simulink library "MCHP_Blockset"  (R2014b)
settings: Solver=ode45  SolverMode=SingleTasking  StartTime=0.0  StopTime=10.0  RelTol=1e-3
InitFcn:
  | disp('MCHP_Blockset_Library_InitFunction');
undefined symbols (not defined in the file): A0, A2, AD0, AVdd, B1, B5, B9, C10, C2, CMP2A, CMP3A, CMP4A, EXTREF1, EXTREF2, gcbh, MaxPer, MCHP_ACC_SAMx_Callback, MCHP_ADC_Callback, MCHP_ADC_HighSpeed_SAR_Callback, MCHP_ADC_HighSpeed_SAR_dsPIC_Callback, MCHP_ADC_SAME5x_Callback, MCHP_AFEC_SAM7x_Callback, MCHP_BUS_I2C_MASTER_callback, MCHP_BUS_SPI_callback, MCHP_C_function_Call_callback, MCHP_CN_Callback, MCHP_COMPARATOR1_callback, MCHP_CompilerOptimisation_Callback, MCHP_DACC_SAMx_Callback, MCHP_Digital_Input_Callback, MCHP_Digital_Output_Read_Callback, MCHP_Digital_Output_Write_Callback, MCHP_Fun, MCHP_HighSpeed_AnalogComparator_Callback, MCHP_IC_Callback, MCHP_IdleTask_Callback, MCHP_Interrupt_Callback, MCHP_Master_Callback, MCHP_MCPWM_Callback, MCHP_MCU_LOAD_Callback, MCHP_MCU_OVERLOAD_Callback, MCHP_MSI_Callback, MCHP_OC_HW_Callback, MCHP_OC_SW_Callback, MCHP_OP_AMP_Callback, MCHP_OrderInOut, MCHP_PDEC_Callback, MCHP_PGA_Callback, MCHP_PWM_Callback, MCHP_PWM_HighSpeed_Override_Callback, MCHP_PWM_HS_FEP_Callback, MCHP_PWM_SAM7x_Callback, MCHP_PWM_SAM7x_Override_Callback, MCHP_QDEC_SAMx_Callback, MCHP_QEI_Callback, MCHP_Scheduler_Options_Callback, MCHP_SECONDARY_CORE_Callback, MCHP_Tasks_State_Callback, MCHP_TCC_PWM_Callback, MCHP_TIMER_Config_Callback ... (+18)
libraries: MCHP_Blockset x2
(part 8 of 9)

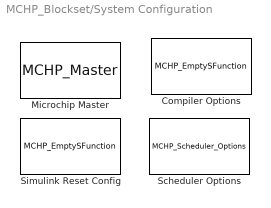
== system MCHP_Blockset/System Configuration ==
  Compiler Options : S-Function  Priority=1  InitFcn=MCHP_CompilerOptimisation_Callback(gcbh, 'InitFcn');  FunctionName=MCHP_EmptySFunction  EnableBusSupport=off  mask{LATEST_CMPLR=on, COMP_LIST=Dynamic Options, COMP_LIST_TXT=Dynamic Options, DFP_LIST=Dynamic Options, DFP_LIST_TXT=Dynamic Options, CMSIS_DSP=Dynamic Options, CMSIS_DSP_TXT=Dynamic Options, USE_64BIT_DOUBLE=off, MCHP_MULTITHREAD_COMPILATION=on, UseCustom_LinkerScript=off, LinkerScript=, MCHP_MASTERLINK=CVLK_SAME70_Modified_CompilerBlock_R2014b/Microchip Master, OPTIMIZATION_LEVEL=2, MPLAB_LINKLIB=default, MPLAB_LINKLIB1=fast floating-point math, CodeReplacement=Dynamic Options, CodeReplacement_TXT=None, OPTIMIZATION_FLTO=off, OPTIMIZATION_REORDER=off, UNROLL_LOOPS=off, PROCEDURAL_ABSTRACTION=off, CUSTOM_OPTIM=, CUSTOM_OPTIM_LD=, MCODE=is less than 32768 (faster), MCONST=in data memory, MDATA=Use only memory below address 8192 (faster), MSCALAR=Use only memory below address 8192 (faster), MLARGEARRAY=off, MAGGREGATE=off, HEAP_SIZE=0, OMF=elf, DEBUG_INFO=on, ProduceHexOutput=off, AssemblyListing=off, SaveTemps=off, NO_EDS_WARN=on, PRINT_STATISTICS=off}
      mask prompts: LATEST_CMPLR "Always use the latest compiler"; COMP_LIST "Select Compiler"; DFP_LIST "Device Family Pack (DFP)"; CMSIS_DSP "CMSIS DSP library"; USE_64BIT_DOUBLE "Use 64-bit double"; MCHP_MULTITHREAD_COMPILATION "Multithread Compilation (faster build)"; UseCustom_LinkerScript "Use a Custom Linker Script"; LinkerScript "Linker Script filename (full path if not in the model folder)"; OPTIMIZATION_LEVEL "Optimisation Level"; MPLAB_LINKLIB "Math Library"; MPLAB_LINKLIB1 "Math Library"; CodeReplacement "Code Replacement"; OPTIMIZATION_FLTO "Enable link-time optimizer"; OPTIMIZATION_REORDER "Allow reordering for ( fcts - variable - asm )"; UNROLL_LOOPS "Unroll Loops (improve speed)"; PROCEDURAL_ABSTRACTION "Procedural abstraction (reduce size)"; CUSTOM_OPTIM "Add custom argument for compiler"; CUSTOM_OPTIM_LD "Add custom argument for linker (coma separated)"; MCODE "Code size"; MCONST "Store Constant"; MDATA "Table data"; MSCALAR "Scalar data"; MLARGEARRAY "Allow array larger than 32K"; MAGGREGATE "Use aggregate data model"; HEAP_SIZE "Heap size"; OMF "Binary format :"; DEBUG_INFO "Generate debugging information"; ProduceHexOutput "Produce hex binary output file (.hex)"; AssemblyListing "Produce assembly listing file (.lst)"; SaveTemps "Save intermediate files (.i .p .s)"; NO_EDS_WARN "Disable eds-warning"; PRINT_STATISTICS "Print some statistics"
      mask init:
      | MCHP_CompilerOptimisation_Callback(gcbh, 'INITIALISATION');
      settings: CopyFcn=MCHP_CompilerOptimisation_Callback(gcbh, 'INITIALISATION');  PreSaveFcn=MCHP_Fun.PreSaveFcn_DynamicOptions(gcbh);  OpenFcn=MCHP_CompilerOptimisation_Callback(gcbh, 'OPEN');
      mask Callback LATEST_CMPLR: MCHP_Fun.BlockUpdate(gcbh);
      mask TypeOptions COMP_LIST: Dynamic Options
      mask Callback COMP_LIST: MCHP_Fun.BlockUpdate(gcbh);
      mask TypeOptions DFP_LIST: Dynamic Options
      mask TypeOptions CMSIS_DSP: Dynamic Options
      mask Callback UseCustom_LinkerScript: MCHP_CompilerOptimisation_Callback(gcbh, 'UseCustom_LinkerScript');
      mask TypeOptions OPTIMIZATION_LEVEL: 0 | 1 | 2 | s | 3
      mask TypeOptions MPLAB_LINKLIB: default | fast floating-point math | relaxed floating-point math
      mask TypeOptions MPLAB_LINKLIB1: default | fast floating-point math
      mask TypeOptions CodeReplacement: Dynamic Options
      mask TypeOptions MCODE: is less than 32768 (faster) | is more than 32768
      mask TypeOptions MCONST: in code memory | in data memory
      mask TypeOptions MDATA: Use only memory below address 8192 (faster) | Can use all available memory
      mask TypeOptions MSCALAR: Use only memory below address 8192 (faster) | Can use all available memory
      mask TypeOptions OMF: elf | coff
      mask Display: MCHP_DrawLogo;disp(['Compiler-Version\n' COMP_LIST_TXT]);
  Microchip Master : S-Function  Priority=1  InitFcn=MCHP_Master_Callback(gcbh,'INIT');  FunctionName=MCHP_Master  EnableBusSupport=off  mask{PICREF=33EP512MU810, PICREF_spd=, TIMESTEP_REF=, BUSYFLAG=Dynamic Options, BUSYFLAG_TXT=, VDD_range=Dynamic Options, VDD_range_TXT=, PWRTEN=Not used, BOREN=High Security Code Protection Enabled, BODENV=2.7V, BORV=Not used, FPWRT=128ms, DSBOREN=Enable ZPBOR during Deep Sleep Mode, DSLPBOR=Not used, MCLRE=Enabled, SMCLR=MCLR pin generates a normal system Reset, PMDL1WAY=Allow only one reconfiguration, RSTPRI=Device will obtain reset instruction from Primary flash, TEMP=Not used, SOSCSRC=Not used, SOSCSEL=Not used, IOL1WAY=Allow only one reconfiguration, ALTVREF=Not used, DISUVREG=Not used, DSSWEN=Not used, LPCFG=Not used, RTCBAT=Not used, VBTBOR=Not used, WUTSEL=Not used, POWERSAVE=off, FNOSC=Fast RC Osc w/Div-by-N (FRCDIV), FPR=ECIO w/ PLL 16x, FOSFPR=HS3 w/PLL 16x, FOS=Primary Oscillator, FRANGE=High Range, OSCILLATOR_SELECT=Internal Fast RC (FRC), OSCILLATOR_SELECT_spd=, QUARTZ=, QUARTZ_spd=, POSCGAIN=2x gain setting, POSCBOOST=Boost the kick start of the oscillator, SOSCGAIN=2x gain setting, SOSCBOOST=Boost the kick start of the oscillator, ACTIV_PLL=off, ACTIV_PLL_spd=, MIPS_DESIRED=, MIPS_DESIRED_spd=, CPUDIV=Divide by 1, FPLLMUL=Not used, FPLLIDIV=8x Divider, POSCFREQ=Not used, POSCMD=Primary Oscillator Disabled, POSCMOD=Primary osc disabled, MIPS=, ACLKCON=Optimized for PWM resolution & ADC conversion speed, ACLKCON_spd=, ACLKCON_Info=, FPLLODIV=32x Divider, PLLKEN=Clock switch to PLL source will wait until the PLL lock signal is valid, FCKSM=Clock Switch Enabled; FSCM Enabled, FCKSMEN=Sw Disabled; Mon Disabled, IESO=Enabled, DSWDTPS=1:2^36, FWDTEN=WDT enabled while device is active and disabled in Sleep; SWDTEN bit disabled, FWDTWINSZ=Window size is 25%, FWPSA=1:512, FWPSA0=1:128, FWPSB=1:16, WDT=Disable, WDTPOST=1:32768, WDTPRE=1:128, WDTPS=1:1048576, WINDIS=Watchdog Timer is in non-Window mode, WWDTEN=Non-Window mode, DSWDTEN=Enable DSWDT during Deep Sleep Mode, DSWDTOSC=Select LPRC as DSWDT Reference clock, FPBDIV=Not used, FSOSCEN=Disable Secondary Oscillator, LPRCSEL=Not used, OSCIOFCN=Not used, OSCIOFNC=general purpose digital I/O pin, LVRCFG=Not used, PLL_96MHZ=Not used, PLL96MHZ=Not used, PLLDIV=Not used, WDTCLK=Not used, WDTCMX=Not used, WDTWIN=Watchdog Window is 25% of WDT period, XTCFG=24-32 MHz crystals, XTBST=Boost the kick-start, APL=Aux Flash Code protect is disabled, APLK=Aux Flash Write Protection or Code Protection is Enabled, AWRP=Aux Flash may be written, BSS=No Boot program Flash segment, BWP=Not used, BWRP=Boot Segment may be written, CP=Protection Disabled, EBS=No Boot EEPROM, ESS=No Segment Data EEPROM, GCP=General Segment Code protect is Disabled, GSS=High Security Code Protection Enabled, GSS0=Not used, GSSK=General Segment Write Protection or Code Protection is Enabled, GWRP=General Segment may be written, PWP=Not used, RBS=No Boot RAM, RSS=No Secure RAM, SSS=No Secure Segment, SWRP=Secure segment may be written, WPCFG=Not used, WPDIS=Not used, WPEND=Not used, WPFP=Not used, ICESEL=Communicate on PGEC1/PGED1, ICS=Communicate on PGEC1 and PGED1, JTAGEN=Disable, COE=Not used, RES=Not used, DEBUG=Debugger is disabled, BACKBUG=Not used, BKBUG=Not used, ALTI2C=I2C mapped to SDA1/SCL1 pins, ALTI2C1=I2C1 mapped to SDA1/SCL1 pins, ALTI2C2=I2C2 mapped to SDA2/SCL2 pins, ALTI2C3=I2C3 mapped to SDA3/SCL3 pins, ALTQIO=QEA1; QEB1; INDX1 are selected as inputs to QEI1, ALTSS1=SS1A is selected as the I/O pin for SPI1, CMPPOL0=Hysteresis is applied to falling edge, CMPPOL1=Hysteresis is applied to falling edge, FCANIO=Not used, FETHIO=Default Ethernet I/O, FMIIEN=MII Enabled, FSRSSEL=Not used, FUSBIDIO=Controlled by the USB Module, FVBUSONIO=Not used, HPOL=PWM module high side output pins have active-high output polarity, HYST0=45 mV Hysteresis, HYST1=45 mV Hysteresis, I2C1SEL=Not used, LPOL=PWM module low side output pins have active-high output polarity, PWMPIN=PWM module pins controlled by PORT register at device Reset, RTCOSC=Not used, UPLLEN=USB PLL Disabled, UPLLIDIV=Not used, ATMOD8=Not used, ALTPMP=Not used, I2C2SEL=Not used, ALTADREF=Not used, ALTCVREF=Not used, PWMLOCK=PWM registers may be written without key sequence, INT_PRIORITY_DMA=0, MCHP_TIMER_REQUEST=, MCHP_TIMER_RESULT=, MCHP_PORT=, MCHP_PLLRegisters=, MCHPVAR=, MCHP_CRC=, BTMODE=Not used, RES1=Not used, PLLSS=Not used, RES2=Not used, ALTCMPI=Not used, BOREN1=Not used, ALTRB6=Not used, RETCFG=Not used, DFMCY=Not used, BSS2=No Boot Segment, BSEN=No Boot Segment, CWRP=Configuration Segment may be written, CSS=No Protection (other than CWRP), AIVTDIS=Disable Alternate Vector Table, BSLIM=Not used, WDTEN=Disable, BTSWP=BOOTSWP instruction is disabled, DBCC=No Cross Connection between DAC outputs, CTXT1=Not Assigned, CTXT2=Not Assigned, SEQNUM=Not used, nSEQNUM=Not used, BOREN0=Enabled, DMTIVT=Not used, DMTCNT=2^8 (256), DMTEN=Dead Man Timer is Disabled and can be enabled by software, ON=Not used, USERID=Not used, RESERVED1=Not used, PGL1WAY=Allow only one reconfiguration, FPLLRNG=34-68 MHz Input, FPLLICLK=FRC is input to the System PLL, FPLLMULT=PLL Multiply by 128, UPLLFSEL=USB PLL input is 24 MHz, DMTINTV=Window/Interval value is 127/128 counter value, WDTSPGM=WDT stops during Flash programming, FDMTEN=Deadman Timer is disabled, TRCEN=Trace features in the CPU are enabled, BOOTISA=Boot code and Exception code is MIPS32, FECCCON=ECC and Dynamic ECC are disabled (ECCCON bits are writable), EXTDDRSIZE=Not used, FSLEEP=Flash is powered down when the device is in Sleep mode, DBGPER=Allow CPU access to all permission regions, EJTAGBEN=Normal EJTAG functionality, TSEQ=Not used, CSEQ=Not used, RWDTPS=1:1048576, RCLKSEL=Always use LPRC, SWDTPS=1:1048576, DMTIVTL=Not used, DMTIVTH=Not used, DMTCNTL=Not used, DMTCNTH=Not used, DMTDIS=Dead Man Timer is Disabled and can be enabled by software, SMBEN=SMBus input threshold is enabled, SPI2PIN=SPI2 uses I/O remap (PPS) pins, CTXT3=Not Assigned, CTXT4=Not Assigned, MBXM0=Mailbox register configured for Master data read (Slave to Master data transfer), MBXM1=Mailbox register configured for Master data read (Slave to Master data transfer), MBXM2=Mailbox register configured for Master data read (Slave to Master data transfer), MBXM3=Mailbox register configured for Master data read (Slave to Master data transfer), MBXM4=Mailbox register configured for Master data read (Slave to Master data transfer), MBXM5=Mailbox register configured for Master data read (Slave to Master data transfer), MBXM6=Mailbox register configured for Master data read (Slave to Master data transfer), MBXM7=Mailbox register configured for Master data read (Slave to Master data transfer), MBXM8=Mailbox register configured for Master data read (Slave to Master data transfer), MBXM9=Mailbox register configured for Master data read (Slave to Master data transfer), MBXM10=Mailbox register configured for Master data read (Slave to Master data transfer), MBXM11=Mailbox register configured for Master data read (Slave to Master data transfer), MBXM12=Mailbox register configured for Master data read (Slave to Master data transfer), MBXM13=Mailbox register configured for Master data read (Slave to Master data transfer), MBXM14=Mailbox register configured for Master data read (Slave to Master data transfer), MBXM15=Mailbox register configured for Master data read (Slave to Master data transfer), MBXHSA=MSIxMBXD15 assigned to mailbox handshake protocol block A, MBXHSB=MSIxMBXD15 assigned to mailbox handshake protocol block B, MBXHSC=MSIxMBXD15 assigned to mailbox handshake protocol block C, MBXHSD=MSIxMBXD15 assigned to mailbox handshake protocol block D, MBXHSE=MSIxMBXD15 assigned to mailbox handshake protocol block E, MBXHSF=MSIxMBXD15 assigned to mailbox handshake protocol block F, MBXHSG=MSIxMBXD15 assigned to mailbox handshake protocol block G, MBXHSH=MSIxMBXD15 assigned to mailbox handshake protocol block H, HSAEN=Mailbox data flow control handshake protocol block disabled, HSBEN=Mailbox data flow control handshake protocol block disabled, HSCEN=Mailbox data flow control handshake protocol block disabled, HSDEN=Mailbox data flow control handshake protocol block disabled, HSEEN=Mailbox data flow control handshake protocol block disabled, HSFEN=Mailbox data flow control handshake protocol block disabled, HSGEN=Mailbox data flow control handshake protocol block disabled, HSHEN=Mailbox data flow control handshake protocol block disabled, CPRA0=Master core owns pin, CPRA1=Master core owns pin, CPRA2=Master core owns pin, CPRA3=Master core owns pin, CPRA4=Master core owns pin, CPRB0=Master core owns pin, CPRB1=Master core owns pin, CPRB2=Master core owns pin, CPRB3=Master core owns pin, CPRB4=Master core owns pin, CPRB5=Master core owns pin, CPRB6=Master core owns pin, CPRB7=Master core owns pin, CPRB8=Master core owns pin, CPRB9=Master core owns pin, CPRB10=Master core owns pin, CPRB11=Master core owns pin, CPRB12=Master core owns pin, CPRB13=Master core owns pin, CPRB14=Master core owns pin, CPRB15=Master core owns pin, CPRC0=Master core owns pin, CPRC1=Master core owns pin, CPRC2=Master core owns pin, CPRC3=Master core owns pin, CPRC4=Master core owns pin, CPRC5=Master core owns pin, CPRC6=Master core owns pin, CPRC7=Master core owns pin, CPRC8=Master core owns pin, CPRC9=Master core owns pin, CPRC10=Master core owns pin, CPRC11=Master core owns pin, CPRC12=Master core owns pin, CPRC13=Master core owns pin, CPRC14=Master core owns pin, CPRC15=Master core owns pin, CPRD0=Master core owns pin, CPRD1=Master core owns pin, CPRD2=Master core owns pin, CPRD3=Master core owns pin, CPRD4=Master core owns pin, CPRD5=Master core owns pin, CPRD6=Master core owns pin, CPRD7=Master core owns pin, CPRD8=Master core owns pin, CPRD9=Master core owns pin, CPRD10=Master core owns pin, CPRD11=Master core owns pin, CPRD12=Master core owns pin, CPRD13=Master core owns pin, CPRD14=Master core owns pin, CPRD15=Master core owns pin, CPRE0=Master core owns pin, CPRE1=Master core owns pin, CPRE2=Master core owns pin, CPRE3=Master core owns pin, CPRE4=Master core owns pin, CPRE5=Master core owns pin, CPRE6=Master core owns pin, CPRE7=Master core owns pin, CPRE8=Master core owns pin, CPRE9=Master core owns pin, CPRE10=Master core owns pin, CPRE11=Master core owns pin, CPRE12=Master core owns pin, CPRE13=Master core owns pin, CPRE14=Master core owns pin, CPRE15=Master core owns pin, S1FNOSC=Internal Fast RC (FRC) Oscillator with postscaler, S1IESO=Start up with FRC; then switch, S1OSCIOFNC=OSC2 is clock output, S1FCKSM=Both Clock switching and Fail-safe Clock Monitor are disabled, S1PLLKEN=S1PLLKEN_ON, S1RWDTPS=1:1048576, S1RCLKSEL=Always use LPRC, S1WINDIS=Watchdog Timer operates in Non-Window mode, S1WDTWIN=WDT Window is 25% of WDT period, S1SWDTPS=1:1048576, S1FWDTEN=use WDTCON.ON bit, S1ICS=Communicate on PGC1 and PGD1, S1DEBUG=Not used, S1ISOLAT=The slave can operate (in debug mode) even if the SLVEN bit in the MSI is zero, S1NOBTSWP=BOOTSWP instruction is disabled, S1ALTI2C1=I2C1 mapped to SDA1/SCL1 pins, S1SPI1PIN=Slave SPI1 uses I/O remap (PPS) pins, S1SSRE=Slave generated resets will reset the Slave Enable Bit in the MSI module, S1MSRE=The master software oriented RESET events (RESET Op-Code; Watchdog timeout; TRAP reset; illegalInstruction) will also cause the slave subsystem to reset, S1CTXT1=Not Assigned, S1CTXT2=Not Assigned, S1CTXT3=Not Assigned, S1CTXT4=Not Assigned, BORLVL=Not used, BSSO=Not used, MCA=Not used, MAXTEMP=Not used, CFGAN14=Not used, CFGAN15=Not used, S1IOL1WAY=Not used, S1BSSO=Not used, S1BACKBUG=Not used, BISTDIS=mBIST on reset feature disabled, NOBTSWP=BOOTSWP instruction is disabled, S1BISTDIS=Slave BIST on reset feature disabled, S1DMTIVTL=Not used, S1DMTIVTH=Not used, S1DMTCNTL=Not used, S1DMTCNTH=Not used, S1DMTDIS=Slave Dead Man Timer is Disabled and can be enabled by software, BSEQ=Not used, IBSEQ=Not used, SMB3EN=SMBus 3.0 input levels, FUSBIDIO2=USBID pin is controlled by the USB2 module, FVBUSIO2=VBUSON pin is controlled by the USB2 module, FUSBIDIO1=USBID pin is controlled by the USB1 module, FVBUSIO1=VBUSON pin is controlled by the USB1 module, VBATBOREN=Enable ZPBOR during VBAT Mode, FDSEN=Enable DSEN bit in DSCON, BORSEL=BOR trip voltage 2.1v (Non-OPAMP deviced operation), POSCFGAIN=Gain is G3, POSCAGCDLY=Settling time = 25ms x AGCRNG, POSCAGCRNG=Range 1x, POSCAGC=Automatic Gain Control for Oscillator, FDBGWP=Not used}
      mask prompts: PICREF "Target (need to apply and RE-OPEN this dialog)"; TIMESTEP_REF "Time-Step synchronisation"; BUSYFLAG "Busy Flag Port"; BUSYFLAG_TXT "Busy Flag Port txt"; VDD_range "Vdd applied. Impact timing characteristics"; VDD_range_TXT "Vdd applied. Impact timing characteristics"; PWRTEN "Power-up Timer Enable"; BOREN "Brown-out Reset Enable"; BODENV "Brown Out Voltage"; BORV "Brown-out Reset Voltage"; FPWRT "Power-on Reset Timer Value"; DSBOREN "Deep Sleep Zero-Power BOR Enable"; DSLPBOR "Deep Sleep Zero-Power BOR Enable"; MCLRE "Master Clear Enable"; SMCLR "Soft Master Clear Enable"; PMDL1WAY "Peripheral Module Disable Configuration"; RSTPRI "Reset Target Vector Select"; TEMP "Temperature Protection Enable"; SOSCSRC "SOSC Source Type"; SOSCSEL "SOSC Power Selection Configuration"; IOL1WAY "Peripheral pin select configuration"; ALTVREF "Alternate VREF location Enable"; DISUVREG "Internal USB 3.3V Regulator Disable"; DSSWEN "DSEN Enable"; LPCFG "Low power regulator control"; RTCBAT "RTC Battery Operation Enable"; VBTBOR "VBAT BOR enable"; WUTSEL "Voltage Regulator Wake-up Time Select"; POWERSAVE "Power Save Mode (Idle)"; FNOSC "Oscillator Source Selection"; FPR "Primary Oscillator Mode"; FOSFPR "Oscillator"; FOS "Oscillator Source"; FRANGE "Frequency Range Select"; OSCILLATOR_SELECT "Oscillator Source"; QUARTZ "Quartz Frequency (Hz)"; POSCGAIN "Primary Oscillator Gain"; POSCBOOST "Primary Oscillator Boost Kick Start"; SOSCGAIN "Secondary Oscillator Gain"; SOSCBOOST "Secondary Oscillator Boost Kick Start"; ACTIV_PLL "Activate clock multiplier/divider (PLL)"; MIPS_DESIRED "Targetted Instructin Per Seconds (IPS in Hz)"; CPUDIV "CPU clock division factor"; FPLLMUL "PLL Multiplier"; FPLLIDIV "PLL Input Divider"; POSCFREQ "Primary Oscillator Frequency Range Configuration"; POSCMD "Primary Oscillator Mode"; POSCMOD "Primary Oscillator Configuration"; ACLKCON "Auxilliary Clock for PWM & ADC"; ACLKCON_Info "Auxilliary Clock Infos:"; FPLLODIV "System PLL Output Clock Divider"; PLLKEN "PLL Lock Enable"; FCKSM "Clock Switching and Monitor"; FCKSMEN "Clock Switching and Monitor"; IESO "Two-speed Oscillator Start-Up"; DSWDTPS "Deep Sleep Watchdog Timer Postscale"; FWDTEN "Watchdog Timer Enable"; FWDTWINSZ "Watchdog Timer Window Size"; FWPSA "WDT Prescaler A"; FWPSA0 "WDT Prescaler"; FWPSB "WDT Prescaler B"; WDT "Watchdog Timer"; WDTPOST "Watchdog Timer Postscaler"; WDTPRE "Watchdog Timer Prescaler"; WDTPS "Watchdog Timer Postscaler"; WINDIS "Watchdog Timer Window"; WWDTEN "Watchdog Timer Window"; DSWDTEN "Deep Sleep Watchdog Timer"; DSWDTOSC "DSWDT Reference Clock Select"; FPBDIV "Peripheral Clock Divisor"; FSOSCEN "Secondary Oscillator Enable"; LPRCSEL "LPRC Oscillator Power and Accuracy"; OSCIOFCN "OSC2 Pin Function"; OSCIOFNC "OSC2 Pin Function"; PLL_96MHZ "96MHz PLL"; PLL96MHZ "96MHz PLL Disable"; PLLDIV "96 MHz PLL Prescaler Select"; WDTCLK "WDT Clock Source Select bits"; WDTCMX "WDT Clock Source Select bits"; WDTWIN "Watch Dog Timer Window Width"; XTCFG "Crystal Oscillator Drive Select depending on crystal value"; XTBST "Oscillator Kick-Start Programmability bit"; APL "Auxiliary Segment Code-protect"; APLK "Auxiliary Segment Key"; AWRP "Auxiliary Segment Write-protect"; BSS "Boot segment Protect"; BWP "Boot Flash Write Protect"; BWRP "Boot Segment Write Protect"; CP "Code Protect"; EBS "Boot Segment Data EEPROM Protection"; ESS "Secure Segment Data EEPROM Protection"; GCP "General Segment Code Protection"; GSS "General Segment Code Protection"; GSS0 "General Segment Code Protect"; GSSK "General Segment Key"; GWRP "General Code Segment Write Protect"; PWP "Program Flash Write Protect"; RBS "Boot Segment Data RAM Protection"; RSS "Secure Segment Data RAM Protection"; SSS "Secure Segment Program Flash Code Protection"; SWRP "Secure Segment Program Write Protect"; WPCFG "Configuration Word Code Page Protection Select"; WPDIS "Segment Write Protection Disable"; WPEND "Segment Write Protection End Page Select"; WPFP "Write Protection Flash Page Segment Boundary"; ICESEL "ICE/ICD Comm Channel Select"; ICS "ICD Communication Channel Select"; JTAGEN "JTAG Port Enable"; COE "Set Clip On Emulation Mode"; RES "Set Clip On Emulation"; DEBUG "Background Debugger Enable"; BACKBUG "Background Debug"; BKBUG "Background Debugger Enable"; ALTI2C "Alternate I2C  pins"; ALTI2C1 "Alternate I2C pins for I2C1"; ALTI2C2 "Alternate I2C pins for I2C2"; ALTI2C3 "Alternate I2C pins for I2C3"; ALTQIO "Enable Alternate QEI1 pin"; ALTSS1 "Enable Alternate SS1 pin"; CMPPOL0 "Comparator Hysteresis Polarity (even comp)"; CMPPOL1 "Comparator Hysteresis Polarity (odd comp)"; FCANIO "CAN I/O Pin Select"; FETHIO "Ethernet I/O Pin Select"; FMIIEN "Ethernet RMII/MII Enable"; FSRSSEL "SRS Select"; FUSBIDIO "USB USID Selection"; FVBUSONIO "USB VBUS ON Selection"; HPOL "Motor Control PWM High Side Polarity"; HYST0 "Even Comparator Hysteresis Select"; HYST1 "Odd Comparator Hysteresis Select"; I2C1SEL "Alternate I2C1 Pin Mapping"; LPOL "Motor Control PWM Low Side Polarity"; PWMPIN "Motor Control PWM Module Pin Mode"; RTCOSC "RTCC Reference Clock Select"; UPLLEN "USB PLL Enable"; UPLLIDIV "USB PLL Input Divider"; ALTPMP "Alternate PMP Pin Mapping"; I2C2SEL "Alternate I2C2"; ALTADREF "External 12-Bit A/D Reference Location"; ALTCVREF "External Comparator Reference Location"; PWMLOCK "PWM Lock Enable"; INT_PRIORITY_DMA "DMA Interrupt Priority"; MCHP_PLLRegisters "MCHP_PLLReg"; BTMODE "xxx"; RES1 "xxx"; PLLSS "PLL Secondary Selection Configuration bit"; ALTCMPI "Alternate Comparator Input bit"; BOREN1 "BOR Override bit"; ALTRB6 "Alternate RB6 pin function enable bit"; RETCFG "xxx"; DFMCY "Data Flash Memory Cycle Count"; BSS2 "Boot Segment Control bit"; BSEN "Boot Segment Control bit"; CWRP "Configuration Segment Write-Protect bit"; CSS "Configuration Segment Code-Protect Level bits"; AIVTDIS "Alternate Interrupt Vector Table bit"; BSLIM "Boot Segment Flash Page Address Limit bits"; WDTEN "Watchdog Timer Enable"; BTSWP "BOOTSWP Instruction Enable/Disable bit"; DBCC "DACx Output Cross Connection bit"; CTXT1 "Specifies Interrupt Priority Level (IPL) Associated to Alternate Working Register 1 bits"; CTXT2 "Specifies Interrupt Priority Level (IPL) Associated to Alternate Working Register 2 bits"; SEQNUM "Sequence Number to Determine the Active Panel in Dual Panel Mode bits"; nSEQNUM "xxx"; BOREN0 "xxx"; DMTIVT "xxx"; DMTCNT "Deadman Timer Count Selection"; DMTEN "Deadman Timer Count Selection"; ON "xxx"; USERID "xxx"; RESERVED1 "xxx"; PGL1WAY "Permission Group Lock One Way Configuration"; FPLLRNG "System PLL Input Range"; FPLLICLK "System PLL Input Clock Selection"; FPLLMULT "System PLL Multiplier"; UPLLFSEL "USB PLL Input Frequency Selection"; DMTINTV "DMT Count Window Interval"; WDTSPGM "Watchdog Timer Stop During Flash Programming"; FDMTEN "Deadman Timer Enable"; TRCEN "Trace Enable"; BOOTISA "Boot ISA Selection"; FECCCON "Dynamic Flash ECC Configuration"; FSLEEP "Flash Sleep Mode"; DBGPER "Debug Mode CPU Access Permission"; EJTAGBEN "EJTAG Boot"; TSEQ "xxx"; CSEQ "xxx"; RWDTPS "Run Mode Watchdog Timer Post Scaler select bits"; RCLKSEL "Watchdog Timer Clock Select bits"; SWDTPS "Sleep Mode Watchdog Timer Post Scaler select bits"; DMTIVTL "xxx"; DMTIVTH "xxx"; DMTCNTL "xxx"; DMTCNTH "xxx"; DMTDIS "Dead Man Timer Disable bit"; SMBEN "SM Bus Enable"; SPI2PIN "SPI2 Pin Select bit"; CTXT3 "Specifies Interrupt Priority Level (IPL) Associated to Alternate Working Register 3 bits"; CTXT4 "Specifies Interrupt Priority Level (IPL) Associated to Alternate Working Register 4 bits"; MBXM0 "Mailbox 0 data direction"; MBXM1 "Mailbox 1 data direction"; MBXM2 "Mailbox 2 data direction"; MBXM3 "Mailbox 3 data direction"; MBXM4 "Mailbox 4 data direction"; MBXM5 "Mailbox 5 data direction"; MBXM6 "Mailbox 6 data direction"; MBXM7 "Mailbox 7 data direction"; MBXM8 "Mailbox 8 data direction"; MBXM9 "Mailbox 9 data direction"; MBXM10 "Mailbox 10 data direction"; MBXM11 "Mailbox 11 data direction"; MBXM12 "Mailbox 12 data direction"; MBXM13 "Mailbox 13 data direction"; MBXM14 "Mailbox 14 data direction"; MBXM15 "Mailbox 15 data direction"; MBXHSA "Mailbox Protocol A assigned to mailbox x"; MBXHSB "Mailbox Protocol B assigned to mailbox x"; MBXHSC "Mailbox Protocol C assigned to mailbox x"; MBXHSD "Mailbox Protocol D assigned to mailbox x"; MBXHSE "Mailbox Protocol E assigned to mailbox x"; MBXHSF "Mailbox Protocol F assigned to mailbox x"; MBXHSG "Mailbox Protocol G assigned to mailbox x"; MBXHSH "Mailbox Protocol H assigned to mailbox x"; HSAEN "Mailbox A data flow control protocol block enable"; HSBEN "Mailbox B data flow control protocol block enable"; HSCEN "Mailbox C data flow control protocol block enable"; HSDEN "Mailbox D data flow control protocol block enable"; HSEEN "Mailbox E data flow control protocol block enable"; HSFEN "Mailbox F data flow control protocol block enable"; HSGEN "Mailbox G data flow control protocol block enable"; HSHEN "Mailbox H data flow control protocol block enable"; CPRA0 "Pin RA0 Ownership Bits"; CPRA1 "Pin RA1 Ownership Bits"; CPRA2 "Pin RA2 Ownership Bits"; CPRA3 "Pin RA3 Ownership Bits"; CPRA4 "Pin RA4 Ownership Bits"; CPRB0 "Pin RB0 Ownership Bits"; CPRB1 "Pin RB1 Ownership Bits"; CPRB2 "Pin RB2 Ownership Bits"; CPRB3 "Pin RB3 Ownership Bits"; CPRB4 "Pin RB4 Ownership Bits"; CPRB5 "Pin RB5 Ownership Bits"; CPRB6 "Pin RB6 Ownership Bits"; CPRB7 "Pin RB7 Ownership Bits"; CPRB8 "Pin RB8 Ownership Bits"; CPRB9 "Pin RB9 Ownership Bits"; CPRB10 "Pin RB10 Ownership Bits"; CPRB11 "Pin RB11 Ownership Bits"; CPRB12 "Pin RB12 Ownership Bits"; CPRB13 "Pin RB13 Ownership Bits"; CPRB14 "Pin RB14 Ownership Bits"; CPRB15 "Pin RB15 Ownership Bits"; CPRC0 "Pin RC0 Ownership Bits"; CPRC1 "Pin RC1 Ownership Bits"; CPRC2 "Pin RC2 Ownership Bits"; CPRC3 "Pin RC3 Ownership Bits"; CPRC4 "Pin RC4 Ownership Bits"; CPRC5 "Pin RC5 Ownership Bits"; CPRC6 "Pin RC6 Ownership Bits"; CPRC7 "Pin RC7 Ownership Bits"; CPRC8 "Pin RC8 Ownership Bits"; CPRC9 "Pin RC9 Ownership Bits"; CPRC10 "Pin RC10 Ownership Bits"; CPRC11 "Pin RC11 Ownership Bits"; CPRC12 "Pin RC12 Ownership Bits"; CPRC13 "Pin RC13 Ownership Bits"; CPRC14 "Pin RC14 Ownership Bits"; CPRC15 "Pin RC15 Ownership Bits"; CPRD0 "Pin RD0 Ownership Bits"; CPRD1 "Pin RD1 Ownership Bits"; CPRD2 "Pin RD2 Ownership Bits"; CPRD3 "Pin RD3 Ownership Bits"; CPRD4 "Pin RD4 Ownership Bits"; CPRD5 "Pin RD5 Ownership Bits"; CPRD6 "Pin RD6 Ownership Bits"; CPRD7 "Pin RD7 Ownership Bits"; CPRD8 "Pin RD8 Ownership Bits"; CPRD9 "Pin RD9 Ownership Bits"; CPRD10 "Pin RD10 Ownership Bits"; CPRD11 "Pin RD11 Ownership Bits"; CPRD12 "Pin RD12 Ownership Bits"; CPRD13 "Pin RD13 Ownership Bits"; CPRD14 "Pin RD14 Ownership Bits"; CPRD15 "Pin RD15 Ownership Bits"; CPRE0 "Pin RE0 Ownership Bits"; CPRE1 "Pin RE1 Ownership Bits"; CPRE2 "Pin RE2 Ownership Bits"; CPRE3 "Pin RE3 Ownership Bits"; CPRE4 "Pin RE4 Ownership Bits"; CPRE5 "Pin RE5 Ownership Bits"; CPRE6 "Pin RE6 Ownership Bits"; CPRE7 "Pin RE7 Ownership Bits"; CPRE8 "Pin RE8 Ownership Bits"; CPRE9 "Pin RE9 Ownership Bits"; CPRE10 "Pin RE10 Ownership Bits"; CPRE11 "Pin RE11 Ownership Bits"; CPRE12 "Pin RE12 Ownership Bits"; CPRE13 "Pin RE13 Ownership Bits"; CPRE14 "Pin RE14 Ownership Bits"; CPRE15 "Pin RE15 Ownership Bits"; S1FNOSC "Oscillator Source Selection"; S1IESO "Two-speed Oscillator Start-Up"; S1OSCIOFNC "Slave OSC2 Pin Function bit"; S1FCKSM "Clock Switching and Monitor"; S1RWDTPS "Run Mode Watchdog Timer Post Scaler select bits"; S1RCLKSEL "Watchdog Timer Clock Select bits"; S1WINDIS "Watchdog Timer Window"; S1WDTWIN "Watchdog Timer Window Select bits"; S1SWDTPS "Sleep Mode Watchdog Timer Post Scaler select bits"; S1FWDTEN "Watchdog Timer Enable"; S1ICS "Slave ICD Communication Channel"; S1DEBUG "Background Debugger Enable"; S1ISOLAT "Isolate the Slave core subsystem from the master subsystem during Debug"; S1NOBTSWP "BOOTSWP Instruction Enable/Disable bit"; S1ALTI2C1 "Alternate I2C1 Pin bit"; S1SPI1PIN "S1 SPI1 Pin Select bit"; S1SSRE "Slave Slave Reset Enable"; S1MSRE "Master Slave Reset Enable"; S1CTXT1 "Specifies Interrupt Priority Level (IPL) Associated to Alternate Working Register 1 bits"; S1CTXT2 "Specifies Interrupt Priority Level (IPL) Associated to Alternate Working Register 2 bits"; S1CTXT3 "Specifies Interrupt Priority Level (IPL) Associated to Alternate Working Register 3 bits"; S1CTXT4 "Specifies Interrupt Priority Level (IPL) Associated to Alternate Working Register 4 bits"; BORLVL "xxx"; BSSO "xxx"; MCA "xxx"; MAXTEMP "xxx"; CFGAN14 "xxx"; CFGAN15 "xxx"; S1IOL1WAY "xxx"; S1BSSO "xxx"; S1BACKBUG "xxx"; BISTDIS "Memory BIST Feature Disable"; NOBTSWP "BOOTSWP instruction disable bit"; S1BISTDIS "Slave BIST on reset disable bit"; S1DMTIVTL "xxx"; S1DMTIVTH "xxx"; S1DMTCNTL "xxx"; S1DMTCNTH "xxx"; S1DMTDIS "Slave Dead Man Timer Disable bit"; BSEQ "xxx"; IBSEQ "xxx"; SMB3EN "SM Bus Enable"; FUSBIDIO2 "USB2 USBID Selection"; FVBUSIO2 "USB2 VBUSON Selection bit"; FUSBIDIO1 "USB1 USBID Selection"; FVBUSIO1 "USB2 VBUSON Selection bit"; VBATBOREN "VBAT BOR Enable"; FDSEN "Deep Sleep Enable"; BORSEL "Brown-out trip voltage"; POSCFGAIN "Primary Oscillator Fine Gain Control bits"; POSCAGCDLY "AGC Gain Search Step Settling Time Control"; POSCAGCRNG "AGC Lock Range bit"; POSCAGC "Primary Oscillator Gain Control bit"; FDBGWP "xxx"
      mask init:
      | MCHP_Master_Callback(gcbh,'INITIALISATION')
      settings: PreSaveFcn=MCHP_Fun.PreSaveFcn_DynamicOptions(gcbh);  OpenFcn=MCHP_Master_Callback(gcbh,'OPEN');
      mask TypeOptions PICREF: Undefined | 30F2010 | 30F2011 | 30F2012 | 30F3010 | 30F3011 | 30F3012 | 30F3013 | 30F3014 | 30F4011 | 30F4012 | 30F4013 | 30F5011 | 30F5013 | 30F5015 | 30F5016 | 30F6010 | 30F6011 | 30F6012 | 30F6013 | 30F6014 | 30F6015 | 33CH128MP202 | 33CH128MP202S1 | 33CH128MP203 | 33CH128MP203S1 | 33CH128MP205 | 33CH128MP205S1 | 33CH128MP206 | 33CH128MP206S1 | 33CH128MP208 | 33CH128MP208S1 | 33CH128MP502 | 33CH128MP502S1 | 33CH128MP503 | 33CH128MP503S1 | 33CH128MP505 | 33CH128MP505S1 | 33CH128MP506 | 33CH128MP506S1 | 33CH128MP508 | 33CH128MP508S1 | 33CH256MP205 | 33CH256MP205S1 | 33CH256MP206 | 33CH256MP206S1 | 33CH256MP208 | 33CH256MP208S1 | 33CH256MP505 | 33CH256MP505S1 | 33CH256MP506 | 33CH256MP506S1 | 33CH256MP508 | 33CH256MP508S1 | 33CH512MP205 | 33CH512MP205S1 | 33CH512MP206 | 33CH512MP206S1 | 33CH512MP208 | 33CH512MP208S1 | 33CH512MP505 | 33CH512MP505S1 | 33CH512MP506 | 33CH512MP506S1 | 33CH512MP508 | 33CH512MP508S1 | 33CH64MP202 | 33CH64MP202S1 | 33CH64MP203 | 33CH64MP203S1 | 33CH64MP205 | 33CH64MP205S1 | 33CH64MP206 | 33CH64MP206S1 | 33CH64MP208 | 33CH64MP208S1 | 33CH64MP502 | 33CH64MP502S1 | 33CH64MP503 | 33CH64MP503S1 | 33CH64MP505 | 33CH64MP505S1 | 33CH64MP506 | 33CH64MP506S1 | 33CH64MP508 | 33CH64MP508S1 | 33CK128MP202 | 33CK128MP203 | 33CK128MP205 | 33CK128MP206 | 33CK128MP208 | 33CK128MP502 | 33CK128MP503 | 33CK128MP505 | 33CK128MP506 | 33CK128MP508 | 33CK256MP202 | 33CK256MP203 | 33CK256MP205 | 33CK256MP206 | 33CK256MP208 | 33CK256MP502 | 33CK256MP503 | 33CK256MP505 | 33CK256MP506 | 33CK256MP508 | 33CK32MP102 | 33CK32MP103 | 33CK32MP105 | 33CK32MP202 | 33CK32MP203 | 33CK32MP205 | 33CK32MP206 | 33CK32MP502 | 33CK32MP503 | 33CK32MP505 | 33CK32MP506 | 33CK64MP102 | 33CK64MP103 | 33CK64MP105 | 33CK64MP202 | 33CK64MP203 | 33CK64MP205 | 33CK64MP206 | 33CK64MP208 | 33CK64MP502 | 33CK64MP503 | 33CK64MP505 | 33CK64MP506 | 33CK64MP508 | 33EP128GM304 | 33EP128GM306 | 33EP128GM310 | 33EP128GM604 | 33EP128GM706 | 33EP128GM710 | 33EP128GP502 | 33EP128GP504 | 33EP128GP506 | 33EP128GS702 | 33EP128GS704 | 33EP128GS705 | 33EP128GS706 | 33EP128GS708 | 33EP128GS804 | 33EP128GS805 | 33EP128GS806 | 33EP128GS808 | 33EP128MC202 | 33EP128MC204 | 33EP128MC206 | 33EP128MC502 | 33EP128MC504 | 33EP128MC506 | 33EP16GS202 | 33EP16GS502 | 33EP16GS504 | 33EP16GS505 | 33EP16GS506 | 33EP256GM304 | 33EP256GM306 | 33EP256GM310 | 33EP256GM604 | 33EP256GM706 | 33EP256GM710 | 33EP256GP502 | 33EP256GP504 | 33EP256GP506 | 33EP256MC202 | 33EP256MC204 | 33EP256MC206 | 33EP256MC502 | 33EP256MC504 | 33EP256MC506 | 33EP256MU806 | 33EP256MU810 | 33EP256MU814 | 33EP32GP502 | 33EP32GP503 | 33EP32GP504 | 33EP32GS202 | 33EP32GS502 | 33EP32GS504 | 33EP32GS505 | 33EP32GS506 | 33EP32MC202 | 33EP32MC203 | 33EP32MC204 | 33EP32MC502 | 33EP32MC503 | 33EP32MC504 | 33EP512GM304 | 33EP512GM306 | 33EP512GM310 | 33EP512GM604 | 33EP512GM706 | 33EP512GM710 | 33EP512GP502 | 33EP512GP504 | 33EP512GP506 | 33EP512GP806 | 33EP512MC202 | 33EP512MC204 | 33EP512MC206 | 33EP512MC502 | 33EP512MC504 | 33EP512MC506 | 33EP512MC806 | 33EP512MU810 | 33EP512MU814 | 33EP64GP502 | 33EP64GP503 | 33EP64GP504 | 33EP64GP506 | 33EP64GS502 | 33EP64GS504 | 33EP64GS505 | 33EP64GS506 | 33EP64GS708 | 33EP64GS804 | 33EP64GS805 | 33EP64GS806 | 33EP64GS808 | 33EP64MC202 | 33EP64MC203 | 33EP64MC204 | 33EP64MC206 | 33EP64MC502 | 33EP64MC503 | 33EP64MC504 | 33EP64MC506 | 33EV128GM002 | 33EV128GM003 | 33EV128GM004 | 33EV128GM006 | 33EV128GM102 | 33EV128GM103 | 33EV128GM104 | 33EV128GM106 | 33EV256GM002 | 33EV256GM003 | 33EV256GM004 | 33EV256GM006 | 33EV256GM102 | 33EV256GM103 | 33EV256GM104 | 33EV256GM106 | 33EV32GM002 | 33EV32GM003 | 33EV32GM004 | 33EV32GM006 | 33EV32GM102 | 33EV32GM103 | 33EV32GM104 | 33EV32GM106 | 33EV64GM002 | 33EV64GM003 | 33EV64GM004 | 33EV64GM006 | 33EV64GM102 | 33EV64GM103 | 33EV64GM104 | 33EV64GM106 | 33FJ06GS001 | 33FJ06GS101 | 33FJ06GS101A | 33FJ06GS102 | 33FJ06GS102A | 33FJ06GS202 | 33FJ06GS202A | 33FJ09GS302 | 33FJ128GP202 | 33FJ128GP204 | 33FJ128GP206 | 33FJ128GP206A | 33FJ128GP306 | 33FJ128GP306A | 33FJ128GP310 | 33FJ128GP310A | 33FJ128GP706 | 33FJ128GP706A | 33FJ128GP708 | 33FJ128GP708A | 33FJ128GP710 | 33FJ128GP710A | 33FJ128GP802 | 33FJ128GP804 | 33FJ128MC202 | 33FJ128MC204 | 33FJ128MC506 | 33FJ128MC506A | 33FJ128MC510 | 33FJ128MC510A | 33FJ128MC706 | 33FJ128MC706A | 33FJ128MC708 | 33FJ128MC708A | 33FJ128MC710 | 33FJ128MC710A | 33FJ128MC802 | 33FJ128MC804 | 33FJ12GP201 | 33FJ12GP202 | 33FJ12MC201 | 33FJ12MC202 | 33FJ16GP304 | 33FJ16GS402 | 33FJ16GS404 | 33FJ16GS502 | 33FJ16GS504 | 33FJ16MC304 | 33FJ256GP506 | 33FJ256GP506A | 33FJ256GP510 | 33FJ256GP510A | 33FJ256GP710 | 33FJ256GP710A | 33FJ256MC510 | 33FJ256MC510A | 33FJ256MC710 | 33FJ256MC710A | 33FJ32GP202 | 33FJ32GP204 | 33FJ32GP302 | 33FJ32GP304 | 33FJ32GS406 | 33FJ32GS606 | 33FJ32GS608 | 33FJ32GS610 | 33FJ32MC202 | 33FJ32MC204 | 33FJ32MC302 | 33FJ32MC304 | 33FJ64GP202 | 33FJ64GP204 | 33FJ64GP206 | 33FJ64GP206A | 33FJ64GP306 | 33FJ64GP306A | 33FJ64GP310 | 33FJ64GP310A | 33FJ64GP706 | 33FJ64GP706A | 33FJ64GP708 | 33FJ64GP708A | 33FJ64GP710 | 33FJ64GP710A | 33FJ64GP802 | 33FJ64GP804 | 33FJ64GS406 | 33FJ64GS606 | 33FJ64GS608 | 33FJ64GS610 | 33FJ64MC202 | 33FJ64MC204 | 33FJ64MC506 | 33FJ64MC506A | 33FJ64MC508 | 33FJ64MC508A | 33FJ64MC510 | 33FJ64MC510A | 33FJ64MC706 | 33FJ64MC706A | 33FJ64MC710 | 33FJ64MC710A | 33FJ64MC802 | 33FJ64MC804 | 32MK0256GPG048 | 32MK0256GPG064 | 32MK0256MCJ048 | 32MK0256MCJ064 | 32MK0512GPG048 | 32MK0512GPG064 | 32MK0512GPK064 | 32MK0512GPK100 | 32MK0512MCF064 | 32MK0512MCF100 | 32MK0512MCJ048 | 32MK0512MCJ064 | 32MK0512MCM064 | 32MK0512MCM100 | 32MK1024GPK064 | 32MK1024GPK100 | 32MK1024MCF064 | 32MK1024MCF100 | 32MK1024MCM064 | 32MK1024MCM100 | 32MZ1024EFG064 | 32MZ1024EFG100 | 32MZ1024EFG124 | 32MZ1024EFG144 | 32MZ1024EFH064 | 32MZ1024EFH100 | 32MZ1024EFH124 | 32MZ1024EFH144 | 32MZ1024EFM064 | 32MZ1024EFM100 | 32MZ1024EFM124 | 32MZ1024EFM144 | 32MZ2048EFG064 | 32MZ2048EFG100 | 32MZ2048EFG124 | 32MZ2048EFG144 | 32MZ2048EFH064 | 32MZ2048EFH100 | 32MZ2048EFH124 | 32MZ2048EFH144 | 32MZ2048EFM064 | 32MZ2048EFM100 | 32MZ2048EFM124 | 32MZ2048EFM144 | PIC32CM1216MC00032 - TQFP32 | PIC32CM1216MC00048 - TQFP48 | PIC32CM6408MC00032 - TQFP32 | PIC32CM6408MC00048 - TQFP48 | SAMC20E15A - QFN32 | SAMC20E16A - QFN32 | SAMC20E17A - QFN32 | SAMC20E18A - QFN32 | SAMC20G15A - QFN48 | SAMC20G16A - QFN48 | SAMC20G17A - QFN48 | SAMC20G18A - QFN48 | SAMC20J15A - QFN64 | SAMC20J16A - QFN64 | SAMC20J17A - QFN64 | SAMC20J17AU - WLCSP56 | SAMC20J18A - QFN64 | SAMC20J18AU - WLCSP56 | SAMC20N17A - QFN100 | SAMC20N18A - QFN100 | SAMC21E15A - QFN32 | SAMC21E16A - QFN32 | SAMC21E17A - QFN32 | SAMC21E18A - QFN32 | SAMC21G15A - QFN48 | SAMC21G16A - QFN48 | SAMC21G17A - QFN48 | SAMC21G18A - QFN48 | SAMC21J15A - QFN64 | SAMC21J16A - QFN64 | SAMC21J17A - QFN64 | SAMC21J17AU - WLCSP56 | SAMC21J18A - TQFP64 | SAMC21J18A - QFN64 | SAMC21J18AU - WLCSP56 | SAMC21N17A - QFN100 | SAMC21N18A - QFN100 | SAMD20E14 - QFN32 | SAMD20E15 - QFN32 | SAMD20E16 - QFN32 | SAMD20E17 - QFN32 | SAMD20E18 - QFN32 | SAMD20E1F - QFN32 | SAMD20G14 - QFN48 | SAMD20G15 - QFN48 | SAMD20G16 - QFN48 | SAMD20G17 - QFN48 | SAMD20G17U - WLCSP45 | SAMD20G18 - QFN48 | SAMD20G18U - WLCSP45 | SAMD20J14 - QFN64 | SAMD20J15 - QFN64 | SAMD20J16 - QFN64 | SAMD20J17 - QFN64 | SAMD20J18 - CTBGA64 | SAMD20J18 - QFN64 | SAMD20E14B - QFN32 | SAMD20E15B - QFN32 | SAMD20E15BU - WLCSP27 | SAMD20E16B - QFN32 | SAMD20E16BU - WLCSP27 | SAMD20G14B - QFN48 | SAMD20G15B - QFN48 | SAMD20G16B - QFN48 | SAMD20J14B - QFN64 | SAMD20J15B - QFN64 | SAMD20J16B - QFN64 | SAMD21E15A - QFN32 | SAMD21E15A - TQFP32 | SAMD21E16A - QFN32 | SAMD21E16A - TQFP32 | SAMD21E17A - QFN32 | SAMD21E17A - TQFP32 | SAMD21E18A - QFN32 | SAMD21E18A - TQFP32 | SAMD21G15A - QFN48 | SAMD21G16A - QFN48 | SAMD21G17A - QFN48 | SAMD21G17AU - WLCSP45 | SAMD21G18A - QFN48 | SAMD21G18AU - WLCSP45 | SAMD21J15A - QFN64 | SAMD21J16A - CTBGA64 | SAMD21J16A - QFN64 | SAMD21J17A - CTBGA64 | SAMD21J17A - QFN64 | SAMD21J18A - CTBGA64 | SAMD21J18A - QFN64 | SAMD21E15B - QFN32 | SAMD21E15BU - WLCSP35 | SAMD21E16B - QFN32 | SAMD21E16BU - WLCSP35 | SAMD21G15B - QFN48 | SAMD21G16B - QFN48 | SAMD21J15B - QFN64 | SAMD21J15B - UFBGA64 | SAMD21J16B - QFN64 | SAMD21J16B - UFBGA64 | SAMD21E15CU - WLCSP35 | SAMD21E16CU - WLCSP35 | SAMD21E17D - QFN32 | SAMD21E17DU - WLCSP35 | SAMD21G17D - QFN48 | SAMD21J17D - QFN64 | SAMD21J17D - CTBGA64 | SAMD21E15L - QFN32 | SAMD21E16L - QFN32 | SAMD21E17L - QFN32 | SAMD21E17L - SOIC32 | SAMD21F17L - SOIC28 | SAMD21G15L - QFN48 | SAMD21G16L - QFN48 | SAMD21G17L - QFN48 | SAME51G18A - QFN48 | SAME51G19A - QFN48 | SAME51J18A - QFN64 | SAME51J19A - QFN64 | SAME51J20A - QFN64 | SAME51N19A - TQFP100 | SAME51N20A - TQFP100 | SAME53J18A - QFN64 | SAME53J19A - QFN64 | SAME53J20A - QFN64 | SAME53N19A - TQFP100 | SAME53N20A - TQFP100 | SAME54N19A - TQFP100 | SAME54N20A - TQFP100 | SAME54P19A - TFBGA120 | SAME54P19A - TQFP128 | SAME54P20A - TFBGA120 | SAME54P20A - TQFP128 | SAME70J19B - LQFP64 | SAME70J20B - LQFP64 | SAME70J21B - LQFP64 | SAME70N19B - TFBGA100 | SAME70N19B - LQFP100 | SAME70N20B - TFBGA100 | SAME70N20B - LQFP100 | SAME70N21B - TFBGA100 | SAME70N21B - LQFP100 | SAME70Q19B - LFBGA144 | SAME70Q19B - UFBGA144 | SAME70Q19B - LQFP144 | SAME70Q20B - LFBGA144 | SAME70Q20B - UFBGA144 | SAME70Q20B - LQFP144 | SAME70Q21B - LFBGA144 | SAME70Q21B - UFBGA144 | SAME70Q21B - LQFP144 | SAMRH71F20B - CQFP256 | SAMRH71F20C - CQFP256 | SAMS70J19B - LQFP64 | SAMS70J19B - QFN64 | SAMS70J20B - LQFP64 | SAMS70J20B - QFN64 | SAMS70J21B - LQFP64 | SAMS70J21B - QFN64 | SAMS70N19B - TFBGA100 | SAMS70N19B - VFBGA100 | SAMS70N19B - LQFP100 | SAMS70N20B - TFBGA100 | SAMS70N20B - VFBGA100 | SAMS70N20B - LQFP100 | SAMS70N21B - TFBGA100 | SAMS70N21B - VFBGA100 | SAMS70N21B - LQFP100 | SAMS70Q19B - LFBGA144 | SAMS70Q19B - UFBGA144 | SAMS70Q19B - LQFP144 | SAMS70Q20B - LFBGA144 | SAMS70Q20B - UFBGA144 | SAMS70Q20B - LQFP144 | SAMS70Q21B - LFBGA144 | SAMS70Q21B - UFBGA144 | SAMS70Q21B - LQFP144 | SAMV70J19B - LQFP64 | SAMV70J20B - LQFP64 | SAMV70N19B - TFBGA100 | SAMV70N19B - LQFP100 | SAMV70N20B - TFBGA100 | SAMV70N20B - LQFP100 | SAMV70Q19B - TFBGA144 | SAMV70Q19B - LQFP144 | SAMV70Q20B - TFBGA144 | SAMV70Q20B - LQFP144 | SAMV71J19B - LQFP64 | SAMV71J20B - LQFP64 | SAMV71J21B - LQFP64 | SAMV71N19B - TFBGA100 | SAMV71N19B - LQFP100 | SAMV71N20B - TFBGA100 | SAMV71N20B - LQFP100 | SAMV71N21B - TFBGA100 | SAMV71N21B - LQFP100 | SAMV71Q19B - TFBGA144 | SAMV71Q19B - LQFP144 | SAMV71Q20B - TFBGA144 | SAMV71Q20B - LQFP144 | SAMV71Q21B - TFBGA144 | SAMV71Q21B - LQFP144
      mask Callback PICREF: MCHP_Master_Callback(gcbh , 'PICREF' ); % do not use spd field as that cause a problem
      mask TypeOptions BUSYFLAG: Dynamic Options
      mask TypeOptions VDD_range: Dynamic Options
      mask TypeOptions PWRTEN: Not used
      mask TypeOptions BOREN: Enabled | Disable | High Security Code Protection Enabled
      mask TypeOptions BODENV: 2.7V | 4.2V | 4.5V | 2.0V
      mask TypeOptions BORV: Not used
      mask TypeOptions FPWRT: 128ms | 64ms | 32ms | 16ms | 8ms | 4ms | 2ms | Off | Timer Disabled | Disable
      mask TypeOptions DSBOREN: Enable ZPBOR during Deep Sleep Mode | Disable ZPBOR during Deep Sleep Mode
      mask TypeOptions DSLPBOR: Not used
      mask TypeOptions MCLRE: Enabled | Disable
      mask TypeOptions SMCLR: MCLR pin generates a normal system Reset | MCLR pin generates an emulated POR Reset
      mask TypeOptions PMDL1WAY: Allow only one reconfiguration | Allow multiple reconfigurations
      mask TypeOptions RSTPRI: Device will obtain reset instruction from Primary flash | Device will obtain reset instruction from Aux flash
      mask TypeOptions TEMP: Not used
      mask TypeOptions SOSCSRC: Not used
      mask TypeOptions SOSCSEL: Not used
      mask TypeOptions IOL1WAY: Allow only one reconfiguration | Allow multiple reconfigurations | Allow Only One Re-configuration | Allow Multiple Re-configurations
      mask TypeOptions ALTVREF: Not used
      mask TypeOptions DISUVREG: Not used
      mask TypeOptions DSSWEN: Not used
      mask TypeOptions LPCFG: Not used
      mask TypeOptions RTCBAT: Not used
      mask TypeOptions VBTBOR: Not used
      mask TypeOptions WUTSEL: Not used
      mask TypeOptions FNOSC: Primary Oscillator (HS; EC) w/ PLL | Primary Oscillator (HS; EC) | Internal Fast RC (FRC) w/ PLL | Internal Fast RC (FRC) | Internal Fast RC (FRC) Oscillator with postscaler | Back up Fast RC (BFRC) Oscillator | Low-Power RC Oscillator (LPRC) | Primary Oscillator with PLL module (XT + PLL; HS + PLL; EC + PLL) | Primary Oscillator (XT; HS; EC) | Fast RC Oscillator with PLL module (FRCPLL) | Fast RC Oscillator with divide-by-N with PLL module (FRCPLL) | Secondary Oscillator (SOSC) | Fast RC Oscillator with divide-by-16 | Internal Fast RC (FRC) Oscillator with divide-by-16 | Primary Oscillator (XT; HS; EC) with PLL | Internal Fast RC with PLL (FRCPLL) | Internal Fast RC (FRC) Oscillator with divide by 16 | Internal Fast RC (FRC) with divide by 16 | Low Power RC oscillator (LPRC) | Internal Fast RC (FRC) with PLL | Internal Fast RC (FRC) oscillator | Internal Fast RC (FRC) with divide by N | Internal Fast RC (FRC) divide by 16 | Primary Oscillator (XT; HS; EC) w/ PLL | Primary Oscillator (MS; HS; EC) w/ PLL | Primary Oscillator (MS; HS; EC) | Low Power RC Osc (LPRC) | Low Power Secondary Osc (SOSC) | USB PLL (UPLL) | Primary Osc (HS;EC) | System PLL | Fast RC Osc w/Div-by-N (FRCDIV)
      mask TypeOptions FPR: ECIO w/ PLL 16x | ECIO w/ PLL 8x | ECIO w/ PLL 4x | ECIO | EC | ERC | ERCIO | XT w/PLL 16x | XT w/PLL 8x | XT w/PLL 4x | XT | HS | XTL | FRC w/ PLL 8x | FRC w/ PLL 16x | FRC w/ PLL 4x
      mask TypeOptions FOSFPR: HS3 w/PLL 16x | HS3 w/PLL 8x | HS3 w/PLL 4x | HS2 w/PLL 16x | HS2 w/PLL 8x | HS2 w/PLL 4x | ECIO w/PLL 16x | ECIO w/PLL 8x | ECIO w/PLL 4x | FRC w/PLL 8x | XT w/PLL 16x | XT w/PLL 8x | XT w/PLL 4x | FRC w/PLL 16x | FRC w/PLL 4x | ECIO | EC | ERC | ERCIO | XT | HS | XTL | Internal Low-Power RC (No change to Primary Osc Mode bits) | Internal Fast RC (No change to Primary Osc Mode bits) | Low-Power 32KHz Osc (No change to Primary Osc Mode bits)
      mask TypeOptions FOS: Primary Oscillator | Internal Low-Power RC | Internal Fast RC | Low-Power 32KHz Osc <TMR1 Osc>
      mask TypeOptions FRANGE: High Range | Low Range
      mask TypeOptions OSCILLATOR_SELECT: Internal Fast RC (FRC) | Internal Fast Low Power RC (LPFRC) | Internal Low Power RC (LPRC) | Crystal / Ceramic resonator | External Clock | Internal Low Power 32 768 Hz Osc | Internal 48MHz Oscillator | Crystal Oscillator at 32kHz on XIN32/XOUT32 | Crystal Oscillator in 8-48MHz on XIN/XOUT 0 | Crystal Oscillator in 8-48MHz on XIN/XOUT 1 | External Clock in 8-48Mhz on XIN 0 | External Clock in 8-48Mhz on XIN 1
      mask Callback OSCILLATOR_SELECT: MCHP_Fun.BlockUpdate(gcbh); % Make sure it is executed at least once! %if ~strcmp(get_param(gcbh , 'OSCILLATOR_SELECT') , get_param(gcbh , 'OSCILLATOR_SELECT_spd')) MCHP_Master_Callback(gcbh , 'OSCILLATOR_SELECT' );  end;
      mask Callback QUARTZ: if ~strcmp(get_param(gcbh , 'QUARTZ'),get_param(gcbh , 'QUARTZ_spd')) MCHP_Fun.BlockUpdate(gcbh);  end;
      mask TypeOptions POSCGAIN: Gain Level 3 (highest) | Gain Level 2 | Gain Level 1 | Gain Level 0 (Lowest) | 2x gain setting | 1.5x gain setting | 1x gain setting | 0.5x gain setting
      mask TypeOptions POSCBOOST: Boost the kick start of the oscillator | Normal start of the oscillator
      mask TypeOptions SOSCGAIN: Gain is G3 | Gain is G2 | Gain is G1 | Gain is G0 | 2x gain setting | 1.5x gain setting | 0.5x gain setting | 1x gain setting | Gain Level 3 (highest) | Gain Level 2 | Gain Level 1 | Gain Level 0 (Lowest)
      mask TypeOptions SOSCBOOST: Boost the kick start of the oscillator | Normal start of the oscillator
      mask Callback ACTIV_PLL: if ~strcmp(get_param(gcbh , 'ACTIV_PLL'),get_param(gcbh , 'ACTIV_PLL_spd')) MCHP_Fun.BlockUpdate(gcbh); end;
      mask Callback MIPS_DESIRED: if ~strcmp(get_param(gcbh , 'MIPS_DESIRED'),get_param(gcbh , 'MIPS_DESIRED_spd')) MCHP_Fun.BlockUpdate(gcbh);  end;
      mask TypeOptions CPUDIV: Divide by 1 | Divide by 2 | Divide by 4 | Divide by 8 | Divide by 16 | Divide by 32 | Divide by 64 | Divide by 128
      mask TypeOptions FPLLMUL: Not used
      mask TypeOptions FPLLIDIV: 8x Divider | 7x Divider | 6x Divider | 5x Divider | 4x Divider | 3x Divider | 2x Divider | 1x Divider
      mask TypeOptions POSCFREQ: Not used
      mask TypeOptions POSCMD: Primary Oscillator Disabled | HS Oscillator Mode | EC Oscillator Mode | HS Crystal Oscillator Mode | XT Crystal Oscillator Mode | EC (External Clock) Mode | XT Oscillator Mode
      mask TypeOptions POSCMOD: Primary Oscillator Disabled | HS Oscillator mode selected | MS Oscillator mode selected | EC Oscillator mode selected | Primary osc disabled | HS osc mode | External clock mode
      mask TypeOptions ACLKCON: Optimized for PWM resolution & ADC conversion speed | Optimized for PWM precision | Optimized for Low Power Consumption | Use Principal Oscillator with PLL | Use Principal Oscillator without PLL | Use FRC with PLL | Use FRC without PLL
      mask Callback ACLKCON: if ~strcmp(get_param(gcbh , 'ACLKCON'),get_param(gcbh , 'ACLKCON_spd')) MCHP_Fun.BlockUpdate(gcbh);  end;
      mask TypeOptions FPLLODIV: 32x Divider | 16x Divider | 8x Divider | 4x Divider | 2x Divider
      mask TypeOptions PLLKEN: PLL lock signal will be used to disable PLL clock output if lock is lost | PLL lock signal is not used; the PLL clock output will not be disabled if lock is lost | PLL clock output will be disabled if LOCK is lost | PLL clock output will not be disabled if LOCK is lost | Clock switch to PLL source will wait until the PLL lock signal is valid | Clock switch will not wait for the PLL lock signal
      mask TypeOptions FCKSM: Sw Disabled; Mon Disabled | Sw Enabled; Mon Disabled | Sw Enabled; Mon Enabled | Both Clock switching and Fail-safe Clock Monitor are disabled | Clock switching is enabled;Fail-safe Clock Monitor is disabled | Both Clock switching and Fail-safe Clock Monitor are enabled | Clock switching and Fail-Safe Clock Monitor are disabled; Mon Disabled | Clock switching is enabled; Fail-Safe Clock Monitor is Disabled | Clock switching and Fail-Safe Clock Monitor are enabled | Clock switching and Fail-Safe Clock Monitor are disabled | Clock switching is enabled; Fail-Safe Clock Monitor is enabled | Clock Switch Enabled; FSCM Enabled | Clock Switch Disabled; FSCM Enabled | Clock Switch Enabled; FSCM Disabled | Clock Switch Disabled; FSCM Disabled
      mask TypeOptions FCKSMEN: Sw Disabled; Mon Disabled | Sw Enabled; Mon Disabled | Sw Enabled; Mon Enabled
      mask TypeOptions IESO: Start up with FRC; then switch | Disable | Start up device with FRC;then automatically switch to user selected oscillator source | Start up device with user selected oscillator source | Enabled
      mask TypeOptions DSWDTPS: 1:2^36 | 1:2^35 | 1:2^34 | 1:2^33 | 1:2^32 | 1:2^31 | 1:2^30 | 1:2^29 | 1:2^28 | 1:2^27 | 1:2^26 | 1:2^25 | 1:2^24 | 1:2^23 | 1:2^22 | 1:2^21 | 1:2^20 | 1:2^19 | 1:2^18 | 1:2^17 | 1:2^16 | 1:2^15 | 1:2^14 | 1:2^13 | 1:2^12 | 1:2^11 | 1:2^10 | 1:2^9 | 1:2^8 | 1:2^7 | 1:2^6 | 1:2^5
      mask TypeOptions FWDTEN: Enable | Disable | WDT controlled via SW; use WDTCON.ON bit | WDT disabled (control is placed on the SWDTEN bit) | WDT enabled while device is active and disabled in Sleep; SWDTEN bit disabled
      mask TypeOptions FWDTWINSZ: Window size is 25% | Window size is 37.5% | Window size is 50% | Window size is 75%
      mask TypeOptions FWPSA: 1:512 | 1:64 | 1:8 | 1:1
      mask TypeOptions FWPSA0: 1:128 | 1:32
      mask TypeOptions FWPSB: 1:16 | 1:15 | 1:14 | 1:13 | 1:12 | 1:11 | 1:10 | 1:9 | 1:8 | 1:7 | 1:6 | 1:5 | 1:4 | 1:3 | 1:2 | 1:1
      mask TypeOptions WDT: Enabled | Disable
      mask TypeOptions WDTPOST: 1:32768 | 1:16;384 | 1:8192 | 1:4096 | 1:2;048 | 1:1024 | 1:512 | 1:256 | 1:128 | 1:64 | 1:32 | 1:16 | 1:8 | 1:4 | 1:2 | 1:1
      mask TypeOptions WDTPRE: 1:128 | 1:32 | Prescaler ratio of 1:128 | Prescaler ratio of 1:32
      mask TypeOptions WDTPS: 1:32768 | 1:16;384 | 1:8192 | 1:4096 | 1:2;048 | 1:1024 | 1:512 | 1:256 | 1:128 | 1:64 | 1:32 | 1:16 | 1:8 | 1:4 | 1:2 | 1:1 | 1:1048576 | 1:524288 | 1:262144 | 1:131072 | 1:65536 | 1:16384 | 1:2048
      mask TypeOptions WINDIS: Watchdog Timer operates in Non-Window mode | Watchdog Timer operates in Window mode | Watchdog Timer in Non-Window mode | Watchdog Timer in Window mode | Watchdog Timer is in non-Window mode | Watchdog Timer is in Window mode
      mask TypeOptions WWDTEN: Non-Window mode | Window mode
      mask TypeOptions DSWDTEN: Enable DSWDT during Deep Sleep Mode | Disable DSWDT during Deep Sleep Mode
      mask TypeOptions DSWDTOSC: Select LPRC as DSWDT Reference clock | Select SOSC as DSWDT Reference Clock
      mask TypeOptions FPBDIV: Not used
      mask TypeOptions FSOSCEN: Enable Secondary Oscillator | Disable Secondary Oscillator
      mask TypeOptions LPRCSEL: Not used
      mask TypeOptions OSCIOFCN: Not used
      mask TypeOptions OSCIOFNC: OSCO pin has clock out function | general purpose digital I/O pin | OSC2 is clock output | Disable | Enabled
      mask TypeOptions LVRCFG: Not used
      mask TypeOptions PLL_96MHZ: Not used
      mask TypeOptions PLL96MHZ: Not used
      mask TypeOptions PLLDIV: Not used
      mask TypeOptions WDTCLK: Not used
      mask TypeOptions WDTCMX: Not used
      mask TypeOptions WDTWIN: WDT Window is 25% of WDT period | WDT Window is 37.5% of WDT period | WDT Window is 50% of WDT period | WDT Windo is 75% of WDT period | WDT Window is 75% of WDT period | Watchdog Window is 25% of WDT period | Watchdog Window is 37.5% of WDT period | Watchdog Window is 50% of WDT period | Watchdog Window is 75% of WDT period
      mask TypeOptions XTCFG: 24-32 MHz crystals | 16-24 MHz crystals | 8-16 MHz crystals | 4-8 MHz crystals
      mask TypeOptions XTBST: Boost the kick-start | Default kick-start
      mask TypeOptions APL: Aux Flash Code protect is disabled | Aux Flash Code protect is enabled
      mask TypeOptions APLK: Aux Flash Write Protection or Code Protection is Enabled | Aux Flash Write Protection and Code Protection is Disabled
      mask TypeOptions AWRP: Aux Flash may be written | Aux Flash is write protected | Auxiliary program memory is not write-protected | Auxiliary program memory is write-protected
      mask TypeOptions BSS: No Boot Segment | Standard Security; Small-sized Boot Flash | Standard Security; Medium-sized Boot Flash | High Security; Small-sized Boot Flash | High Security; Medium-sized Boot Flash | Standard Security; Large-sized Boot Flash | High Security; Large-sized Boot Flash | No Protection (other than BWRP) | Standard Security | High Security | No Boot Segment Program Memory | No Boot program Flash segment
      mask TypeOptions BWP: Not used
      mask TypeOptions BWRP: Boot Segment may be written | Boot Segment is write protected | Boot Segment Program Memory may be written | Boot Segment Program Memory is write protected | Boot segment is write-protected
      mask TypeOptions CP: Protection Disabled | Protection Enabled
      mask TypeOptions EBS: No Boot EEPROM | Boot EEPROM Enabled
      mask TypeOptions ESS: No Segment Data EEPROM | Small-sized Secure Data EEPROM | Medium-sized Secure Data EEPROM | Large-sized Secure Data EEPROM
      mask TypeOptions GCP: Disable | Enabled | High Security Code Protection Enabled | General Segment Code protect is Disabled | General Segment Code protection Enabled | Standard Security Code protection Enabled
      mask TypeOptions GSS: Disable | Enabled | High Security Code Protection Enabled | No Protection (other than GWRP) | Standard Security | High Security | General Segment Code protect is Disabled | Standard Security Code protection Enabled
      mask TypeOptions GSS0: Not used
      mask TypeOptions GSSK: General Segment Write Protection or Code Protection is Enabled | General Segment Write Protection and Code Protection is Disabled
      mask TypeOptions GWRP: General Segment may be written | General Segment is write protected | Disable | Enabled | User program memory is write-protected | Writes to program memory are allowed | Writes to program memory are disabled
      mask TypeOptions PWP: Not used
      mask TypeOptions RBS: No Boot RAM | Small-sized Boot RAM | Medium-sized Boot RAM | Large-sized Boot RAM
      mask TypeOptions RSS: No Secure RAM | Small-sized Secure RAM | Medium-sized Secure RAM | Large-sized Secure RAM
      mask TypeOptions SSS: No Secure Segment | Standard Security; Small-sized Secure Flash | Standard Security; Medium-sized Secure Flash | Standard Security; Large-sized Secure Flash | High Security; Small-sized Secure Flash | High Security; Medium-sized Secure Flash | High Security; Large-sized Secure Flash
      mask TypeOptions SWRP: Disable | Enabled | Secure segment may be written | Secure segment is write protected
      mask TypeOptions WPCFG: Not used
      mask TypeOptions WPDIS: Not used
      mask TypeOptions WPEND: Not used
      mask TypeOptions WPFP: Not used
      mask TypeOptions ICESEL: Communicate on PGEC1/PGED1 | Communicate on PGEC2/PGED2 | Communicate on PGEC3/PGED3
      mask TypeOptions ICS: Use PGC/EMUC and PGD/EMUD | Use EMUC1 and EMUD1 | Use EMUC2 and EMUD2 | Use EMUC3 and EMUD3 | Communicate on PGC1 and PGD1 | Communicate on PGC2 and PGD2 | Communicate on PGC3 and PGD3 | Communicate on PGEC1 and PGED1 | Communicate on PGEC2 and PGED2 | Communicate on PGEC3 and PGED3 | Communicate on PGEC1/PGED1 | Communicate on PGEC2/PGED2 | Communicate on PGEC3/PGED3
      mask TypeOptions JTAGEN: Enable | Disable
      mask TypeOptions COE: Not used
      mask TypeOptions RES: Not used
      mask TypeOptions DEBUG: Debugger is disabled | Debugger is enabled
      mask TypeOptions BACKBUG: Not used
      mask TypeOptions BKBUG: Not used
      mask TypeOptions ALTI2C: I2C mapped to SDA1/SCL1 pins | I2C mapped to ASDA1/ASCL1 pins | I2C mapped to SDA1/SCL1 | I2C mapped to ASDA1/ASCL1
      mask TypeOptions ALTI2C1: I2C1 mapped to SDA1/SCL1 pins | I2C1 mapped to ASDA1/ASCL1 pins | SDA1/SCK1 pins are selected as the I/O pins for I2C1 | ASDA1/ASCK1 pins are selected as the I/O pins for I2C1
      mask TypeOptions ALTI2C2: I2C2 mapped to SDA2/SCL2 pins | I2C2 mapped to ASDA2/ASCL2 pins | SDA2/SCK2 pins are selected as the I/O pins for I2C2 | ASDA2/ASCK2 pins are selected as the I/O pins for I2C2
      mask TypeOptions ALTI2C3: I2C3 mapped to SDA3/SCL3 pins | I2C3 mapped to ASDA3/ASCL3 pins
      mask TypeOptions ALTQIO: QEA1; QEB1; INDX1 are selected as inputs to QEI1 | AQEA1; AQEB1; and AINDX1 are selected as inputs to QEI1
      mask TypeOptions ALTSS1: SS1A is selected as the I/O pin for SPI1 | SS1 is selected as the I/O pin for SPI1
      mask TypeOptions CMPPOL0: Hysteresis is applied to falling edge | Hysteresis is applied to rising edge
      mask TypeOptions CMPPOL1: Hysteresis is applied to falling edge | Hysteresis is applied to rising edge
      mask TypeOptions FCANIO: Not used
      mask TypeOptions FETHIO: Default Ethernet I/O | Alternate Ethernet I/O
      mask TypeOptions FMIIEN: MII Enabled | RMII Enabled
      mask TypeOptions FSRSSEL: Not used
      mask TypeOptions FUSBIDIO: Controlled by the USB Module | Controlled by Port Function
      mask TypeOptions FVBUSONIO: Not used
      mask TypeOptions HPOL: Active High | Active Low | PWM module high side output pins have active-high output polarity | PWM module high side output pins have active-low output polarity
      mask TypeOptions HYST0: 45 mV Hysteresis | 30 mV Hysteresis | 15 mV Hysteresis | No Hysteresis
      mask TypeOptions HYST1: 45 mV Hysteresis | 30 mV Hysteresis | 15 mV Hysteresis | No Hysteresis
      mask TypeOptions I2C1SEL: Not used
      mask TypeOptions LPOL: Active High | Active Low | PWM module low side output pins have active-high output polarity | PWM module low side output pins have active-low output polarity
      mask TypeOptions PWMPIN: Control with PORT/TRIS regs | Control with HPOL/LPOL bits | PWM module pins controlled by PORT register at device Reset | PWM module pins controlled by PWM module at device Reset
      mask TypeOptions RTCOSC: Not used
      mask TypeOptions UPLLEN: USB PLL Disabled | USB PLL Enabled
      mask TypeOptions UPLLIDIV: Not used
      mask TypeOptions ATMOD8: Not used
      mask TypeOptions ALTPMP: Not used
      mask TypeOptions I2C2SEL: Not used
      mask TypeOptions ALTADREF: Not used
      mask TypeOptions ALTCVREF: Not used
      mask TypeOptions PWMLOCK: Certain PWM registers may only be written after key sequence | PWM registers may be written without key sequence
      mask TypeOptions INT_PRIORITY_DMA: 0 | 1 | 2 | 3 | 4 | 5 | 6 | 7
      mask TypeOptions BTMODE: Not used
      mask TypeOptions RES1: Not used
      mask TypeOptions PLLSS: Not used
      mask TypeOptions RES2: Not used
      mask TypeOptions ALTCMPI: Not used
      mask TypeOptions BOREN1: Not used
      mask TypeOptions ALTRB6: Not used
      mask TypeOptions RETCFG: Not used
      mask TypeOptions DFMCY: Not used
      mask TypeOptions BSS2: No Boot Segment | Boot Segment size determined by FBSLIM
      mask TypeOptions BSEN: No Boot Segment | Boot Segment size determined by FBSLIM
      mask TypeOptions CWRP: Configuration Segment may be written | Configuration Segment is write protected
      mask TypeOptions CSS: No Protection (other than CWRP) | Standard Security | Enhanced Security | High Security
      mask TypeOptions AIVTDIS: Disabled AIVT | Enabled AIVT | Disable Alternate Vector Table | Enable Alternate Vector Table
      mask TypeOptions BSLIM: Not used
      mask TypeOptions WDTEN: Enable | WDT disabled (control is placed on the SWDTEN bit) | WDT enabled while device is active and disabled in Sleep; SWDTEN bit disabled | Disable
      mask TypeOptions BTSWP: BOOTSWP instruction is disabled | BOOTSWP instruction is enabled
      mask TypeOptions DBCC: No Cross Connection between DAC outputs | Interconnects DACOUT1 and DACOUT2
      mask TypeOptions CTXT1: Not Assigned | Alternate Register set assigned to IPL level 7 | Alternate Register set assigned to IPL level 6 | Alternate Register set assigned to IPL level 5 | Alternate Register set assigned to IPL level 4 | Alternate Register set assigned to IPL level 3 | Alternate Register set assigned to IPL level 2 | Alternate Register set assigned to IPL level 1 | Alternate register set 1 assigned to IPL level 7 | Alternate register set 1 assigned to IPL level 6 | Alternate register set 1 assigned to IPL level 5 | Alternate register set 1 assigned to IPL level 4 | Alternate register set 1 assigned to IPL level 3 | Alternate register set 1 assigned to IPL level 2 | Alternate register set 1 assigned to IPL level 1
      mask TypeOptions CTXT2: Not Assigned | Alternate Register set assigned to IPL level 7 | Alternate Register set assigned to IPL level 6 | Alternate Register set assigned to IPL level 5 | Alternate Register set assigned to IPL level 4 | Alternate Register set assigned to IPL level 3 | Alternate Register set assigned to IPL level 2 | Alternate Register set assigned to IPL level 1 | Alternate register set 2 assigned to IPL level 7 | Alternate register set 2  assigned to IPL level 6 | Alternate register set 2  assigned to IPL level 5 | Alternate register set 2  assigned to IPL level 4 | Alternate register set 2  assigned to IPL level 3 | Alternate register set 2  assigned to IPL level 2 | Alternate register set 2  assigned to IPL level 1
      mask TypeOptions SEQNUM: Not used
      mask TypeOptions nSEQNUM: Not used
      mask TypeOptions BOREN0: Enabled | Disable
      mask TypeOptions DMTIVT: Not used
      mask TypeOptions DMTCNT: 2^31 (2147483648) | 2^30 (1073741824) | 2^29 (536870912) | 2^28 (268435456) | 2^27 (134217728) | 2^26 (67108864) | 2^25 (33554432) | 2^24 (16777216) | 2^23 (8388608) | 2^22 (4194304) | 2^21 (2097152) | 2^20 (1048576) | 2^19 (524288) | 2^18 (262144) | 2^17 (131072) | 2^16 (65536) | 2^15 (32768) | 2^14 (16384) | 2^13 (8192) | 2^12 (4096) | 2^11 (2048) | 2^10 (1024) | 2^9 (512) | 2^8 (256)
      mask TypeOptions DMTEN: Dead Man Timer is Enabled and cannot be disabled by software | Dead Man Timer is Disabled and can be enabled by software
      mask TypeOptions ON: Not used
      mask TypeOptions USERID: Not used
      mask TypeOptions RESERVED1: Not used
      mask TypeOptions PGL1WAY: Allow only one reconfiguration | Allow multiple reconfigurations
      mask TypeOptions FPLLRNG: 54-64 MHz Input | 34-64 MHz Input | 21-42 MHz Input | 13-26 MHz Input | 8-16 MHz Input | 5-10 MHz Input | Bypass | 34-68 MHz Input
      mask TypeOptions FPLLICLK: FRC is input to the System PLL | POSC is input to the System PLL
      mask TypeOptions FPLLMULT: PLL Multiply by 128 | PLL Multiply by 127 | PLL Multiply by 126 | PLL Multiply by 125 | PLL Multiply by 124 | PLL Multiply by 123 | PLL Multiply by 122 | PLL Multiply by 121 | PLL Multiply by 120 | PLL Multiply by 119 | PLL Multiply by 118 | PLL Multiply by 117 | PLL Multiply by 116 | PLL Multiply by 115 | PLL Multiply by 114 | PLL Multiply by 113 | PLL Multiply by 112 | PLL Multiply by 111 | PLL Multiply by 110 | PLL Multiply by 109 | PLL Multiply by 108 | PLL Multiply by 107 | PLL Multiply by 106 | PLL Multiply by 105 | PLL Multiply by 104 | PLL Multiply by 103 | PLL Multiply by 102 | PLL Multiply by 101 | PLL Multiply by 100 | PLL Multiply by 99 | PLL Multiply by 98 | PLL Multiply by 97 | PLL Multiply by 96 | PLL Multiply by 95 | PLL Multiply by 94 | PLL Multiply by 93 | PLL Multiply by 92 | PLL Multiply by 91 | PLL Multiply by 90 | PLL Multiply by 89 | PLL Multiply by 88 | PLL Multiply by 87 | PLL Multiply by 86 | PLL Multiply by 85 | PLL Multiply by 84 | PLL Multiply by 83 | PLL Multiply by 82 | PLL Multiply by 81 | PLL Multiply by 80 | PLL Multiply by 79 | PLL Multiply by 78 | PLL Multiply by 77 | PLL Multiply by 76 | PLL Multiply by 75 | PLL Multiply by 74 | PLL Multiply by 73 | PLL Multiply by 72 | PLL Multiply by 71 | PLL Multiply by 70 | PLL Multiply by 69 | PLL Multiply by 68 | PLL Multiply by 67 | PLL Multiply by 66 | PLL Multiply by 65 | PLL Multiply by 64 | PLL Multiply by 63 | PLL Multiply by 62 | PLL Multiply by 61 | PLL Multiply by 60 | PLL Multiply by 59 | PLL Multiply by 58 | PLL Multiply by 57 | PLL Multiply by 56 | PLL Multiply by 55 | PLL Multiply by 54 | PLL Multiply by 53 | PLL Multiply by 52 | PLL Multiply by 51 | PLL Multiply by 50 | PLL Multiply by 49 | PLL Multiply by 48 | PLL Multiply by 47 | PLL Multiply by 46 | PLL Multiply by 45 | PLL Multiply by 44 | PLL Multiply by 43 | PLL Multiply by 42 | PLL Multiply by 41 | PLL Multiply by 40 | PLL Multiply by 39 | PLL Multiply by 38 | PLL Multiply by 37 | PLL Multiply by 36 | PLL Multiply by 35 | PLL Multiply by 34 | PLL Multiply by 33 | PLL Multiply by 32 | PLL Multiply by 31 | PLL Multiply by 30 | PLL Multiply by 29 | PLL Multiply by 28 | PLL Multiply by 27 | PLL Multiply by 26 | PLL Multiply by 25 | PLL Multiply by 24 | PLL Multiply by 23 | PLL Multiply by 22 | PLL Multiply by 21 | PLL Multiply by 20 | PLL Multiply by 19 | PLL Multiply by 18 | PLL Multiply by 17 | PLL Multiply by 16 | PLL Multiply by 15 | PLL Multiply by 14 | PLL Multiply by 13 | PLL Multiply by 12 | PLL Multiply by 11 | PLL Multiply by 10 | PLL Multiply by 9 | PLL Multiply by 8 | PLL Multiply by 7 | PLL Multiply by 6 | PLL Multiply by 5 | PLL Multiply by 4 | PLL Multiply by 3 | PLL Multiply by 2 | PLL Multiply by 1
      mask TypeOptions UPLLFSEL: USB PLL input is 24 MHz | USB PLL input is 12 MHz
      mask TypeOptions DMTINTV: Window/Interval value is 127/128 counter value | Window/Interval value is 63/64 counter value | Window/Interval value is 31/32 counter value | Window/Interval value is 15/16 counter value | Window/Interval value is 7/8 counter value | Window/Interval value is 3/4 counter value | Window/Interval value is 1/2 counter value | Window/Interval value is zero
      mask TypeOptions WDTSPGM: WDT stops during Flash programming | WDT runs during Flash programming
      mask TypeOptions FDMTEN: Deadman Timer is enabled | Deadman Timer is disabled
      mask TypeOptions TRCEN: Trace features in the CPU are enabled | Trace features in the CPU are disabled
      mask TypeOptions BOOTISA: Boot code and Exception code is MIPS32 | Boot code and Exception code is microMIPS
      mask TypeOptions FECCCON: ECC and Dynamic ECC are disabled (ECCCON<1:0> bits are writable) | ECC and Dynamic ECC are disabled (ECCCON<1:0> bits are locked) | Dynamic Flash ECC is enabled (ECCCON<1:0> bits are locked) | Flash ECC is enabled (ECCCON<1:0> bits are locked; disables word Flash writes) | ECC and Dynamic ECC are disabled (ECCCON bits are writable) | ECC and Dynamic ECC are disabled (ECCCON bits are locked) | Dynamic Flash ECC is enabled (ECCCON bits are locked) | Flash ECC is enabled (ECCCON bits are locked)
      mask TypeOptions EXTDDRSIZE: Not used
      mask TypeOptions FSLEEP: Flash is powered down when the device is in Sleep mode | Flash power down is controlled by the VREGS bit
      mask TypeOptions DBGPER: Allow CPU access to all permission regions | PG0: Deny PG1: Allow PG2: Allow | PG0: Allow PG1: Deny PG2: Allow | Allow CPU access to Permission Group 2 permission regions | PG0: Allow PG1: Allow PG2: Deny | Allow CPU access to Permission Group 1 permission regions | Allow CPU access to Permission Group 0 permission regions | Deny CPU access to all permission regions
      mask TypeOptions EJTAGBEN: Normal EJTAG functionality | Reduced EJTAG functionality
      mask TypeOptions TSEQ: Not used
      mask TypeOptions CSEQ: Not used
      mask TypeOptions RWDTPS: 1:1048576 | 1:524288 | 1:262144 | 1:131072 | 1:65536 | 1:32768 | 1:16384 | 1:8192 | 1:4096 | 1:2048 | 1:1024 | 1:512 | 1:256 | 1:128 | 1:64 | 1:32 | 1:16 | 1:8 | 1:4 | 1:2 | 1:1 | 1:2147483648 | 1:1073741824 | 1:536870912 | 1:268435456 | 1:134217728 | 1:67108864 | 1:33554432 | 1:16777216 | 1:8388608 | 1:4194304 | 1:2097152
      mask TypeOptions RCLKSEL: Always use LPRC | Use FRC when WINDIS = 0; system clock is not INTOSC/LPRC and device is not in Sleep;otherwise; use INTOSC/LPRC | Use peripheral clk when system clock is not INTOSC/LPRC and device is not in Sleep;otherwise; use INTOSC/LPRC | Always use BFRC/256 | Use FRC when WINDIS = 0 and device is not in Sleep; otherwise; use BFRC/256 | Use peripheral clk when device is not in Sleep; otherwise; use BFRC/256
      mask TypeOptions SWDTPS: 1:1048576 | 1:524288 | 1:262144 | 1:131072 | 1:65536 | 1:32768 | 1:16384 | 1:8192 | 1:4096 | 1:2048 | 1:1024 | 1:512 | 1:256 | 1:128 | 1:64 | 1:32 | 1:16 | 1:8 | 1:4 | 1:2 | 1:1 | 1:2147483648 | 1:1073741824 | 1:536870912 | 1:268435456 | 1:134217728 | 1:67108864 | 1:33554432 | 1:16777216 | 1:8388608 | 1:4194304 | 1:2097152
      mask TypeOptions DMTIVTL: Not used
      mask TypeOptions DMTIVTH: Not used
      mask TypeOptions DMTCNTL: Not used
      mask TypeOptions DMTCNTH: Not used
      mask TypeOptions DMTDIS: Dead Man Timer is Disabled and can be enabled by software | Dead Man Timer is Enabled and cannot be disabled by software
      mask TypeOptions SMBEN: SMBus input threshold is enabled | Standard I2C input threshold operation
      mask TypeOptions SPI2PIN: SPI2 uses I/O remap (PPS) pins | SPI2 uses dedicated I/O pins
      mask TypeOptions CTXT3: Not Assigned | Alternate Register set assigned to IPL level 7 | Alternate Register set assigned to IPL level 6 | Alternate Register set assigned to IPL level 5 | Alternate Register set assigned to IPL level 4 | Alternate Register set assigned to IPL level 3 | Alternate Register set assigned to IPL level 2 | Alternate Register set assigned to IPL level 1
      mask TypeOptions CTXT4: Not Assigned | Alternate Register set assigned to IPL level 7 | Alternate Register set assigned to IPL level 6 | Alternate Register set assigned to IPL level 5 | Alternate Register set assigned to IPL level 4 | Alternate Register set assigned to IPL level 3 | Alternate Register set assigned to IPL level 2 | Alternate Register set assigned to IPL level 1
      mask TypeOptions MBXM0: Mailbox register configured for Master data read (Slave to Master data transfer) | Mailbox register configured for Master data write (Master to Slave data transfer)
      mask TypeOptions MBXM1: Mailbox register configured for Master data read (Slave to Master data transfer) | Mailbox register configured for Master data write (Master to Slave data transfer)
      mask TypeOptions MBXM2: Mailbox register configured for Master data read (Slave to Master data transfer) | Mailbox register configured for Master data write (Master to Slave data transfer)
      mask TypeOptions MBXM3: Mailbox register configured for Master data read (Slave to Master data transfer) | Mailbox register configured for Master data write (Master to Slave data transfer)
      mask TypeOptions MBXM4: Mailbox register configured for Master data read (Slave to Master data transfer) | Mailbox register configured for Master data write (Master to Slave data transfer)
      mask TypeOptions MBXM5: Mailbox register configured for Master data read (Slave to Master data transfer) | Mailbox register configured for Master data write (Master to Slave data transfer)
      mask TypeOptions MBXM6: Mailbox register configured for Master data read (Slave to Master data transfer) | Mailbox register configured for Master data write (Master to Slave data transfer)
      mask TypeOptions MBXM7: Mailbox register configured for Master data read (Slave to Master data transfer) | Mailbox register configured for Master data write (Master to Slave data transfer)
      mask TypeOptions MBXM8: Mailbox register configured for Master data read (Slave to Master data transfer) | Mailbox register configured for Master data write (Master to Slave data transfer)
      mask TypeOptions MBXM9: Mailbox register configured for Master data read (Slave to Master data transfer) | Mailbox register configured for Master data write (Master to Slave data transfer)
      mask TypeOptions MBXM10: Mailbox register configured for Master data read (Slave to Master data transfer) | Mailbox register configured for Master data write (Master to Slave data transfer)
      mask TypeOptions MBXM11: Mailbox register configured for Master data read (Slave to Master data transfer) | Mailbox register configured for Master data write (Master to Slave data transfer)
      mask TypeOptions MBXM12: Mailbox register configured for Master data read (Slave to Master data transfer) | Mailbox register configured for Master data write (Master to Slave data transfer)
      mask TypeOptions MBXM13: Mailbox register configured for Master data read (Slave to Master data transfer) | Mailbox register configured for Master data write (Master to Slave data transfer)
      mask TypeOptions MBXM14: Mailbox register configured for Master data read (Slave to Master data transfer) | Mailbox register configured for Master data write (Master to Slave data transfer)
      mask TypeOptions MBXM15: Mailbox register configured for Master data read (Slave to Master data transfer) | Mailbox register configured for Master data write (Master to Slave data transfer)
      mask TypeOptions MBXHSA: MSIxMBXD15 assigned to mailbox handshake protocol block A | MSIxMBXD14 assigned to mailbox handshake protocol block A | MSIxMBXD13 assigned to mailbox handshake protocol block A | MSIxMBXD12 assigned to mailbox handshake protocol block A | MSIxMBXD11 assigned to mailbox handshake protocol block A | MSIxMBXD10 assigned to mailbox handshake protocol block A | MSIxMBXD9 assigned to mailbox handshake protocol block A | MSIxMBXD8 assigned to mailbox handshake protocol block A | MSIxMBXD7 assigned to mailbox handshake protocol block A | MSIxMBXD6 assigned to mailbox handshake protocol block A | MSIxMBXD5 assigned to mailbox handshake protocol block A | MSIxMBXD4 assigned to mailbox handshake protocol block A | MSIxMBXD3 assigned to mailbox handshake protocol block A | MSIxMBXD2 assigned to mailbox handshake protocol block A | MSIxMBXD1 assigned to mailbox handshake protocol block A | MSIxMBXD0 assigned to mailbox handshake protocol block A
      mask TypeOptions MBXHSB: MSIxMBXD15 assigned to mailbox handshake protocol block B | MSIxMBXD14 assigned to mailbox handshake protocol block B | MSIxMBXD13 assigned to mailbox handshake protocol block B | MSIxMBXD12 assigned to mailbox handshake protocol block B | MSIxMBXD11 assigned to mailbox handshake protocol block B | MSIxMBXD10 assigned to mailbox handshake protocol block B | MSIxMBXD9 assigned to mailbox handshake protocol block B | MSIxMBXD8 assigned to mailbox handshake protocol block B | MSIxMBXD7 assigned to mailbox handshake protocol block B | MSIxMBXD6 assigned to mailbox handshake protocol block B | MSIxMBXD5 assigned to mailbox handshake protocol block B | MSIxMBXD4 assigned to mailbox handshake protocol block B | MSIxMBXD3 assigned to mailbox handshake protocol block B | MSIxMBXD2 assigned to mailbox handshake protocol block B | MSIxMBXD1 assigned to mailbox handshake protocol block B | MSIxMBXD0 assigned to mailbox handshake protocol block B
      mask TypeOptions MBXHSC: MSIxMBXD15 assigned to mailbox handshake protocol block C | MSIxMBXD14 assigned to mailbox handshake protocol block C | MSIxMBXD13 assigned to mailbox handshake protocol block C | MSIxMBXD12 assigned to mailbox handshake protocol block C | MSIxMBXD11 assigned to mailbox handshake protocol block C | MSIxMBXD10 assigned to mailbox handshake protocol block C | MSIxMBXD9 assigned to mailbox handshake protocol block C | MSIxMBXD8 assigned to mailbox handshake protocol block C | MSIxMBXD7 assigned to mailbox handshake protocol block C | MSIxMBXD6 assigned to mailbox handshake protocol block C | MSIxMBXD5 assigned to mailbox handshake protocol block C | MSIxMBXD4 assigned to mailbox handshake protocol block C | MSIxMBXD3 assigned to mailbox handshake protocol block C | MSIxMBXD2 assigned to mailbox handshake protocol block C | MSIxMBXD1 assigned to mailbox handshake protocol block C | MSIxMBXD0 assigned to mailbox handshake protocol block C
      mask TypeOptions MBXHSD: MSIxMBXD15 assigned to mailbox handshake protocol block D | MSIxMBXD14 assigned to mailbox handshake protocol block D | MSIxMBXD13 assigned to mailbox handshake protocol block D | MSIxMBXD12 assigned to mailbox handshake protocol block D | MSIxMBXD11 assigned to mailbox handshake protocol block D | MSIxMBXD10 assigned to mailbox handshake protocol block D | MSIxMBXD9 assigned to mailbox handshake protocol block D | MSIxMBXD8 assigned to mailbox handshake protocol block D | MSIxMBXD7 assigned to mailbox handshake protocol block D | MSIxMBXD6 assigned to mailbox handshake protocol block D | MSIxMBXD5 assigned to mailbox handshake protocol block D | MSIxMBXD4 assigned to mailbox handshake protocol block D | MSIxMBXD3 assigned to mailbox handshake protocol block D | MSIxMBXD2 assigned to mailbox handshake protocol block D | MSIxMBXD1 assigned to mailbox handshake protocol block D | MSIxMBXD0 assigned to mailbox handshake protocol block D
      mask TypeOptions MBXHSE: MSIxMBXD15 assigned to mailbox handshake protocol block E | MSIxMBXD14 assigned to mailbox handshake protocol block E | MSIxMBXD13 assigned to mailbox handshake protocol block E | MSIxMBXD12 assigned to mailbox handshake protocol block E | MSIxMBXD11 assigned to mailbox handshake protocol block E | MSIxMBXD10 assigned to mailbox handshake protocol block E | MSIxMBXD9 assigned to mailbox handshake protocol block E | MSIxMBXD8 assigned to mailbox handshake protocol block E | MSIxMBXD7 assigned to mailbox handshake protocol block E | MSIxMBXD6 assigned to mailbox handshake protocol block E | MSIxMBXD5 assigned to mailbox handshake protocol block E | MSIxMBXD4 assigned to mailbox handshake protocol block E | MSIxMBXD3 assigned to mailbox handshake protocol block E | MSIxMBXD2 assigned to mailbox handshake protocol block E | MSIxMBXD1 assigned to mailbox handshake protocol block E | MSIxMBXD0 assigned to mailbox handshake protocol block E
      mask TypeOptions MBXHSF: MSIxMBXD15 assigned to mailbox handshake protocol block F | MSIxMBXD14 assigned to mailbox handshake protocol block F | MSIxMBXD13 assigned to mailbox handshake protocol block F | MSIxMBXD12 assigned to mailbox handshake protocol block F | MSIxMBXD11 assigned to mailbox handshake protocol block F | MSIxMBXD10 assigned to mailbox handshake protocol block F | MSIxMBXD9 assigned to mailbox handshake protocol block F | MSIxMBXD8 assigned to mailbox handshake protocol block F | MSIxMBXD7 assigned to mailbox handshake protocol block F | MSIxMBXD6 assigned to mailbox handshake protocol block F | MSIxMBXD5 assigned to mailbox handshake protocol block F | MSIxMBXD4 assigned to mailbox handshake protocol block F | MSIxMBXD3 assigned to mailbox handshake protocol block F | MSIxMBXD2 assigned to mailbox handshake protocol block F | MSIxMBXD1 assigned to mailbox handshake protocol block F | MSIxMBXD0 assigned to mailbox handshake protocol block F
      mask TypeOptions MBXHSG: MSIxMBXD15 assigned to mailbox handshake protocol block G | MSIxMBXD14 assigned to mailbox handshake protocol block G | MSIxMBXD13 assigned to mailbox handshake protocol block G | MSIxMBXD12 assigned to mailbox handshake protocol block G | MSIxMBXD11 assigned to mailbox handshake protocol block G | MSIxMBXD10 assigned to mailbox handshake protocol block G | MSIxMBXD9 assigned to mailbox handshake protocol block G | MSIxMBXD8 assigned to mailbox handshake protocol block G | MSIxMBXD7 assigned to mailbox handshake protocol block G | MSIxMBXD6 assigned to mailbox handshake protocol block G | MSIxMBXD5 assigned to mailbox handshake protocol block G | MSIxMBXD4 assigned to mailbox handshake protocol block G | MSIxMBXD3 assigned to mailbox handshake protocol block G | MSIxMBXD2 assigned to mailbox handshake protocol block G | MSIxMBXD1 assigned to mailbox handshake protocol block G | MSIxMBXD0 assigned to mailbox handshake protocol block G
      mask TypeOptions MBXHSH: MSIxMBXD15 assigned to mailbox handshake protocol block H | MSIxMBXD14 assigned to mailbox handshake protocol block H | MSIxMBXD13 assigned to mailbox handshake protocol block H | MSIxMBXD12 assigned to mailbox handshake protocol block H | MSIxMBXD11 assigned to mailbox handshake protocol block H | MSIxMBXD10 assigned to mailbox handshake protocol block H | MSIxMBXD9 assigned to mailbox handshake protocol block H | MSIxMBXD8 assigned to mailbox handshake protocol block H | MSIxMBXD7 assigned to mailbox handshake protocol block H | MSIxMBXD6 assigned to mailbox handshake protocol block H | MSIxMBXD5 assigned to mailbox handshake protocol block H | MSIxMBXD4 assigned to mailbox handshake protocol block H | MSIxMBXD3 assigned to mailbox handshake protocol block H | MSIxMBXD2 assigned to mailbox handshake protocol block H | MSIxMBXD1 assigned to mailbox handshake protocol block H | MSIxMBXD0 assigned to mailbox handshake protocol block H
      mask TypeOptions HSAEN: Mailbox data flow control handshake protocol block disabled | Mailbox data flow control handshake protocol block enabled
      mask TypeOptions HSBEN: Mailbox data flow control handshake protocol block disabled | Mailbox data flow control handshake protocol block enabled
      mask TypeOptions HSCEN: Mailbox data flow control handshake protocol block disabled | Mailbox data flow control handshake protocol block enabled
      mask TypeOptions HSDEN: Mailbox data flow control handshake protocol block disabled | Mailbox data flow control handshake protocol block enabled
      mask TypeOptions HSEEN: Mailbox data flow control handshake protocol block disabled | Mailbox data flow control handshake protocol block enabled
      mask TypeOptions HSFEN: Mailbox data flow control handshake protocol block disabled | Mailbox data flow control handshake protocol block enabled
      mask TypeOptions HSGEN: Mailbox data flow control handshake protocol block disabled | Mailbox data flow control handshake protocol block enabled
      mask TypeOptions HSHEN: Mailbox data flow control handshake protocol block disabled | Mailbox data flow control handshake protocol block enabled
      mask TypeOptions CPRA0: Master core owns pin | Slave 1 core owns pin
      mask TypeOptions CPRA1: Master core owns pin | Slave 1 core owns pin
      mask TypeOptions CPRA2: Master core owns pin | Slave 1 core owns pin
      mask TypeOptions CPRA3: Master core owns pin | Slave 1 core owns pin
      mask TypeOptions CPRA4: Master core owns pin | Slave 1 core owns pin
      mask TypeOptions CPRB0: Master core owns pin | Slave 1 core owns pin
      mask TypeOptions CPRB1: Master core owns pin | Slave 1 core owns pin
      mask TypeOptions CPRB2: Master core owns pin | Slave 1 core owns pin
      mask TypeOptions CPRB3: Master core owns pin | Slave 1 core owns pin
      mask TypeOptions CPRB4: Master core owns pin | Slave 1 core owns pin
      mask TypeOptions CPRB5: Master core owns pin | Slave 1 core owns pin
      mask TypeOptions CPRB6: Master core owns pin | Slave 1 core owns pin
      mask TypeOptions CPRB7: Master core owns pin | Slave 1 core owns pin
      mask TypeOptions CPRB8: Master core owns pin | Slave 1 core owns pin
      mask TypeOptions CPRB9: Master core owns pin | Slave 1 core owns pin
      mask TypeOptions CPRB10: Master core owns pin | Slave 1 core owns pin
      mask TypeOptions CPRB11: Master core owns pin | Slave 1 core owns pin
      mask TypeOptions CPRB12: Master core owns pin | Slave 1 core owns pin
      mask TypeOptions CPRB13: Master core owns pin | Slave 1 core owns pin
      mask TypeOptions CPRB14: Master core owns pin | Slave 1 core owns pin
      mask TypeOptions CPRB15: Master core owns pin | Slave 1 core owns pin
      mask TypeOptions CPRC0: Master core owns pin | Slave 1 core owns pin
      mask TypeOptions CPRC1: Master core owns pin | Slave 1 core owns pin
      mask TypeOptions CPRC2: Master core owns pin | Slave 1 core owns pin
      mask TypeOptions CPRC3: Master core owns pin | Slave 1 core owns pin
      mask TypeOptions CPRC4: Master core owns pin | Slave 1 core owns pin
      mask TypeOptions CPRC5: Master core owns pin | Slave 1 core owns pin
      mask TypeOptions CPRC6: Master core owns pin | Slave 1 core owns pin
      mask TypeOptions CPRC7: Master core owns pin | Slave 1 core owns pin
      mask TypeOptions CPRC8: Master core owns pin | Slave 1 core owns pin
      mask TypeOptions CPRC9: Master core owns pin | Slave 1 core owns pin
      mask TypeOptions CPRC10: Master core owns pin | Slave 1 core owns pin
      mask TypeOptions CPRC11: Master core owns pin | Slave 1 core owns pin
      mask TypeOptions CPRC12: Master core owns pin | Slave 1 core owns pin
      mask TypeOptions CPRC13: Master core owns pin | Slave 1 core owns pin
      mask TypeOptions CPRC14: Master core owns pin | Slave 1 core owns pin
      mask TypeOptions CPRC15: Master core owns pin | Slave 1 core owns pin
      mask TypeOptions CPRD0: Master core owns pin | Slave 1 core owns pin
      mask TypeOptions CPRD1: Master core owns pin | Slave 1 core owns pin
      mask TypeOptions CPRD2: Master core owns pin | Slave 1 core owns pin
      mask TypeOptions CPRD3: Master core owns pin | Slave 1 core owns pin
      mask TypeOptions CPRD4: Master core owns pin | Slave 1 core owns pin
      mask TypeOptions CPRD5: Master core owns pin | Slave 1 core owns pin
      mask TypeOptions CPRD6: Master core owns pin | Slave 1 core owns pin
      mask TypeOptions CPRD7: Master core owns pin | Slave 1 core owns pin
      mask TypeOptions CPRD8: Master core owns pin | Slave 1 core owns pin
      mask TypeOptions CPRD9: Master core owns pin | Slave 1 core owns pin
      mask TypeOptions CPRD10: Master core owns pin | Slave 1 core owns pin
      mask TypeOptions CPRD11: Master core owns pin | Slave 1 core owns pin
      mask TypeOptions CPRD12: Master core owns pin | Slave 1 core owns pin
      mask TypeOptions CPRD13: Master core owns pin | Slave 1 core owns pin
      mask TypeOptions CPRD14: Master core owns pin | Slave 1 core owns pin
      mask TypeOptions CPRD15: Master core owns pin | Slave 1 core owns pin
      mask TypeOptions CPRE0: Master core owns pin | Slave 1 core owns pin
      mask TypeOptions CPRE1: Master core owns pin | Slave 1 core owns pin
      mask TypeOptions CPRE2: Master core owns pin | Slave 1 core owns pin
      mask TypeOptions CPRE3: Master core owns pin | Slave 1 core owns pin
      mask TypeOptions CPRE4: Master core owns pin | Slave 1 core owns pin
      mask TypeOptions CPRE5: Master core owns pin | Slave 1 core owns pin
      mask TypeOptions CPRE6: Master core owns pin | Slave 1 core owns pin
      mask TypeOptions CPRE7: Master core owns pin | Slave 1 core owns pin
      mask TypeOptions CPRE8: Master core owns pin | Slave 1 core owns pin
      mask TypeOptions CPRE9: Master core owns pin | Slave 1 core owns pin
      mask TypeOptions CPRE10: Master core owns pin | Slave 1 core owns pin
      mask TypeOptions CPRE11: Master core owns pin | Slave 1 core owns pin
      mask TypeOptions CPRE12: Master core owns pin | Slave 1 core owns pin
      mask TypeOptions CPRE13: Master core owns pin | Slave 1 core owns pin
      mask TypeOptions CPRE14: Master core owns pin | Slave 1 core owns pin
      mask TypeOptions CPRE15: Master core owns pin | Slave 1 core owns pin
      mask TypeOptions S1FNOSC: Internal Fast RC (FRC) Oscillator with postscaler | Back up Fast RC (BFRC) Oscillator | Low-Power RC Oscillator (LPRC) | Primary Oscillator with PLL module (XT + PLL; HS + PLL; EC + PLL) | Primary Oscillator (XT; HS; EC) | Fast RC Oscillator with divide-by-N with PLL module (FRCPLL) | Internal Fast RC (FRC)
      mask TypeOptions S1IESO: Start up with FRC; then switch | Disable
      mask TypeOptions S1OSCIOFNC: OSC2 is clock output | general purpose digital I/O pin
      mask TypeOptions S1FCKSM: Both Clock switching and Fail-safe Clock Monitor are disabled | Clock switching is enabled;Fail-safe Clock Monitor is disabled | Both Clock switching and Fail-safe Clock Monitor are enabled
      mask TypeOptions S1PLLKEN: S1PLLKEN_ON | S1PLLKEN_OFF
      mask TypeOptions S1RWDTPS: 1:1048576 | 1:524288 | 1:262144 | 1:131072 | 1:65536 | 1:32768 | 1:16384 | 1:8192 | 1:4096 | 1:2048 | 1:1024 | 1:512 | 1:256 | 1:128 | 1:64 | 1:32 | 1:16 | 1:8 | 1:4 | 1:2 | 1:1
      mask TypeOptions S1RCLKSEL: Always use LPRC | Use FRC when WINDIS = 0; system clock is not INTOSC/LPRC and device is not in Sleep; otherwise; use INTOSC/LPRC | Use peripheral clk when system clock is not INTOSC/LPRC and device is not in Sleep;otherwise; use INTOSC/LPRC
      mask TypeOptions S1WINDIS: Watchdog Timer operates in Non-Window mode | Watchdog Timer operates in Window mode
      mask TypeOptions S1WDTWIN: WDT Window is 25% of WDT period | WDT Window is 37.5% of WDT period | WDT Window is 50% of WDT period | WDT Windo is 75% of WDT period
      mask TypeOptions S1SWDTPS: 1:1048576 | 1:524288 | 1:262144 | 1:131072 | 1:65536 | 1:32768 | 1:16384 | 1:8192 | 1:4096 | 1:2048 | 1:1024 | 1:512 | 1:256 | 1:128 | 1:64 | 1:32 | 1:16 | 1:8 | 1:4 | 1:2 | 1:1
      mask TypeOptions S1FWDTEN: Enable | use WDTCON.ON bit
      mask TypeOptions S1ICS: Communicate on PGC1 and PGD1 | Communicate on PGC2 and PGD2 | Communicate on PGC3 and PGD3
      mask TypeOptions S1DEBUG: Not used
      mask TypeOptions S1ISOLAT: The slave can operate (in debug mode) even if the SLVEN bit in the MSI is zero | The slave can only operate if the SLVEN bit in the MSI is set
      mask TypeOptions S1NOBTSWP: BOOTSWP instruction is disabled | BOOTSWP instruction is enabled
      mask TypeOptions S1ALTI2C1: I2C1 mapped to SDA1/SCL1 pins | I2C1 mapped to ASDA1/ASCL1 pins
      mask TypeOptions S1SPI1PIN: Slave SPI1 uses I/O remap (PPS) pins | Slave SPI1 uses dedicated I/O pins
      mask TypeOptions S1SSRE: Slave generated resets will reset the Slave Enable Bit in the MSI module | Slave generated resets will not reset the Slave Enable Bit in the MSI module
      mask TypeOptions S1MSRE: The master software oriented RESET events (RESET Op-Code; Watchdog timeout; TRAP reset; illegalInstruction) will also cause the slave subsystem to reset | The master software oriented RESET events (RESET Op-Code; Watchdog timeout; TRAP reset; illegalInstruction) will not cause the slave subsystem to reset
      mask TypeOptions S1CTXT1: Not Assigned | Alternate Register set assigned to IPL level 7 | Alternate Register set assigned to IPL level 6 | Alternate Register set assigned to IPL level 5 | Alternate Register set assigned to IPL level 4 | Alternate Register set assigned to IPL level 3 | Alternate Register set assigned to IPL level 2 | Alternate Register set assigned to IPL level 1
      mask TypeOptions S1CTXT2: Not Assigned | Alternate Register set assigned to IPL level 7 | Alternate Register set assigned to IPL level 6 | Alternate Register set assigned to IPL level 5 | Alternate Register set assigned to IPL level 4 | Alternate Register set assigned to IPL level 3 | Alternate Register set assigned to IPL level 2 | Alternate Register set assigned to IPL level 1
      mask TypeOptions S1CTXT3: Not Assigned | Alternate Register set assigned to IPL level 7 | Alternate Register set assigned to IPL level 6 | Alternate Register set assigned to IPL level 5 | Alternate Register set assigned to IPL level 4 | Alternate Register set assigned to IPL level 3 | Alternate Register set assigned to IPL level 2 | Alternate Register set assigned to IPL level 1
      mask TypeOptions S1CTXT4: Not Assigned | Alternate Register set assigned to IPL level 7 | Alternate Register set assigned to IPL level 6 | Alternate Register set assigned to IPL level 5 | Alternate Register set assigned to IPL level 4 | Alternate Register set assigned to IPL level 3 | Alternate Register set assigned to IPL level 2 | Alternate Register set assigned to IPL level 1
      mask TypeOptions BORLVL: Not used
      mask TypeOptions BSSO: Not used
      mask TypeOptions MCA: Not used
      mask TypeOptions MAXTEMP: Not used
      mask TypeOptions CFGAN14: Not used
      mask TypeOptions CFGAN15: Not used
      mask TypeOptions S1IOL1WAY: Not used
      mask TypeOptions S1BSSO: Not used
      mask TypeOptions S1BACKBUG: Not used
      mask TypeOptions BISTDIS: mBIST on reset feature disabled | mBIST on reset feature enabled
      mask TypeOptions NOBTSWP: BOOTSWP instruction is disabled | BOOTSWP instruction is enabled
      mask TypeOptions S1BISTDIS: Slave BIST on reset feature disabled | Slave BIST on reset feature enabled
      mask TypeOptions S1DMTIVTL: Not used
      mask TypeOptions S1DMTIVTH: Not used
      mask TypeOptions S1DMTCNTL: Not used
      mask TypeOptions S1DMTCNTH: Not used
      mask TypeOptions S1DMTDIS: Slave Dead Man Timer is Disabled and can be enabled by software | Slave Dead Man Timer is Enabled and cannot be disabled by software
      mask TypeOptions BSEQ: Not used
      mask TypeOptions IBSEQ: Not used
      mask TypeOptions SMB3EN: SMBus 3.0 input levels | Normal  SMBus input levels
      mask TypeOptions FUSBIDIO2: USBID pin is controlled by the USB2 module | USBID pin is controlled by the port function
      mask TypeOptions FVBUSIO2: VBUSON pin is controlled by the USB2 module | VBUSON pin is controlled by the port function
      mask TypeOptions FUSBIDIO1: USBID pin is controlled by the USB1 module | USBID pin is controlled by the port function
      mask TypeOptions FVBUSIO1: VBUSON pin is controlled by the USB1 module | VBUSON pin is controlled by the port function
      mask TypeOptions VBATBOREN: Enable ZPBOR during VBAT Mode | Disable ZPBOR during VBAT Mode
      mask TypeOptions FDSEN: Enable DSEN bit in DSCON | Disable DSEN bit in DSCON
      mask TypeOptions BORSEL: BOR trip voltage 2.1v (Non-OPAMP deviced operation) | BOR trip voltage 2.8v (OPAMP deviced operation)
      mask TypeOptions POSCFGAIN: Gain is G3 | Gain is G2 | Gain is G1 | Gain is G0
      mask TypeOptions POSCAGCDLY: Settling time = 25ms x AGCRNG | Settling time = 6.25ms x AGCRNG | Settling time = 400ms x AGCRNG | Settling time = 100ms x AGCRNG
      mask TypeOptions POSCAGCRNG: Range 1x | Range 5x
      mask TypeOptions POSCAGC: Automatic Gain Control for Oscillator | Manual Gain Control of Oscillator
      mask TypeOptions FDBGWP: Not used
      mask Display: MCHP_DrawLogo;fprintf('MCHP MASTER\\n%s\\n%3.2f MIPS',PICREF,str2num(MIPS)/1e6);
  Scheduler Options : S-Function  InitFcn=MCHP_Scheduler_Options_Callback(gcbh,'InitFcn');  FunctionName=MCHP_Scheduler_Options  Parameters=[],[],[],[],[],-1,0  EnableBusSupport=off  mask(Scheduler Options){TaskOverloadBehaviour=Queue the task (queue length is 1), MCHP_MASTERLINK=UTester_33EP512MU810_CPUOverLoad/Microchip Master}
      mask prompts: TaskOverloadBehaviour "On sub-task Overload:"
      mask help:
      | Scheduler Options apply only to Multi-Tasking implementation (typically Multirate model)
      |
      | - Queue the task:
      | The task is queued and will execute after higher or equal priority task. Higher tasks rate are not impacted. Lower tasks rate are delayed.
      |
      | - Drop this task execution once:
      | The task is dropped. Higher tasks rate are not impacted. Lower tasks rate might execute within the time free up.
      |
      | - Delay all new tasks until end of overload
      | All new tasks execution is delayed including higher tasks rate. Lower tasks rate are delayed but executed. Ratio between tasks rate is kept constant, but average tasks rate is lowered.
      mask init:
      | MCHP_Scheduler_Options_Callback(gcbh,'INITIALISATION');
      settings: CopyFcn=MCHP_Scheduler_Options_Callback(gcbh,'CopyFcn');  OpenFcn=MCHP_Scheduler_Options_Callback(gcbh,'OPEN');
      mask TypeOptions TaskOverloadBehaviour: Queue the task (queue length is 1) | Skip this task execution once | Delay all new tasks until end of overload
      mask Display: MCHP_DrawLogo;disp('Scheduler Options\nQueue');
  Simulink Reset Config : S-Function  FunctionName=MCHP_EmptySFunction  EnableBusSupport=off  mask{MCHP_MASTERLINK=0}
      settings: CopyFcn=MCHP_Simulink_Reset_Config_Callback(gcbh,'COPY');  OpenFcn=MCHP_Simulink_Reset_Config_Callback(gcbh,'OPEN');
      mask Display:
      | MCHP_DrawLogo;
      | disp('Simulink Reset\nConfig');
